simulink model "SR26"  (R2025a)
settings: Solver=FixedStepDiscrete  StartTime=0.0  StopTime=100  FixedStep=0.01  RelTol=1e-3  EnableMultiTasking=on
PreLoadFcn:
  | try, model_open; catch, disp('Error occurred while executing model pre-load callback: model_open.m'); disp('Please assure that the MATLAB working directory is set to the model directory before opening.'); end
InitFcn:
  | try, model_open; catch, end
values from neighbouring files (symbols this model uses):
  dt = 10.0    [SR26.sldd]
undefined symbols (not defined in the file or in its folder): BMSInputProcessing, GCM, raptor_get_safe_string, raptor_xcp_function, RegenEnable, StateCAN, Subsystem, TCEnable
libraries: Utilities x263, Raptor_lib x137, simulink x7, IO x5, APPS_BSPC x4, TorqueCommand x3, Cooling x3, StateMachine x2, DriveSpeed x2, ATCC x2, BrakePressure x2, ThrottlePosition x2
(part 3 of 4)

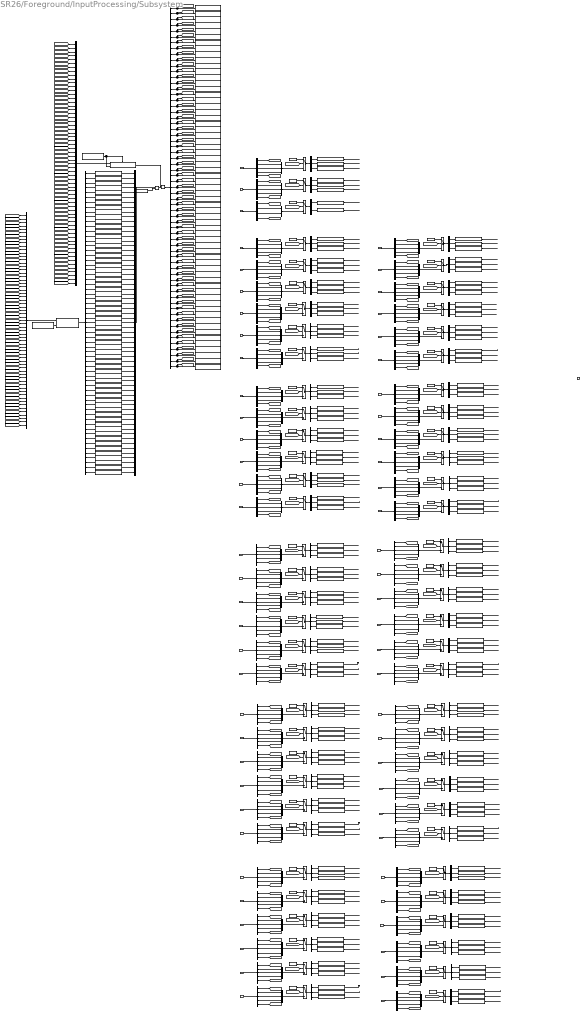
== system SR26/Foreground/InputProcessing/Subsystem ==
  note: Module5
  note: Module4
  note: Module3
  note: Module2
  note: 'IN_module2Cell4V_V'
  note: Module1
  note: times out after 200ms
  IO_CAN2_500_Bus : Inport
  IO_CAN2_501_Bus : Inport  Port=2
  IO_CAN2_502_Bus : Inport  Port=3
  IO_CAN2_503_Bus : Inport  Port=4
  IO_CAN2_504_Bus : Inport  Port=5
  IO_CAN2_505_Bus : Inport  Port=6
  IO_CAN2_506_Bus : Inport  Port=7
  IO_CAN2_507_Bus : Inport  Port=8
  IO_CAN2_508_Bus : Inport  Port=9
  IO_CAN2_509_Bus : Inport  Port=10
  IO_CAN2_510_Bus : Inport  Port=11
  IO_CAN2_511_Bus : Inport  Port=12
  IO_CAN2_512_Bus : Inport  Port=13
  IO_CAN2_513_Bus : Inport  Port=14
  IO_CAN2_514_Bus : Inport  Port=15
  IO_CAN2_515_Bus : Inport  Port=16
  IO_CAN2_516_Bus : Inport  Port=17
  IO_CAN2_517_Bus : Inport  Port=18
  IO_CAN2_518_Bus : Inport  Port=19
  IO_CAN2_519_Bus : Inport  Port=20
  IO_CAN2_520_Bus : Inport  Port=21
  IO_CAN2_521_Bus : Inport  Port=22
  IO_CAN2_522_Bus : Inport  Port=23
  IO_CAN2_523_Bus : Inport  Port=24
  IO_CAN2_524_Bus : Inport  Port=25
  IO_CAN2_525_Bus : Inport  Port=26
  IO_CAN2_526_Bus : Inport  Port=27
  IO_CAN2_527_Bus : Inport  Port=28
  IO_CAN2_528_Bus : Inport  Port=29
  IO_CAN2_529_Bus : Inport  Port=30
  IO_CAN2_530_Bus : Inport  Port=31
  IO_CAN2_531_Bus : Inport  Port=32
  IO_CAN2_532_Bus : Inport  Port=33
  IO_CAN2_533_Bus : Inport  Port=34
  IO_CAN2_534_Bus : Inport  Port=35
  IO_CAN2_535_Bus : Inport  Port=36
  IO_CAN2_536_Bus : Inport  Port=37
  IO_CAN2_537_Bus : Inport  Port=38
  IO_CAN2_538_Bus : Inport  Port=39
  IO_CAN2_539_Bus : Inport  Port=40
  IO_CAN2_540_Bus : Inport  Port=41
  IO_CAN2_541_Bus : Inport  Port=42
  IO_CAN2_542_Bus : Inport  Port=43
  IO_CAN2_543_Bus : Inport  Port=44
  IO_CAN2_544_Bus : Inport  Port=45
  IO_CAN2_545_Bus : Inport  Port=46
  IO_CAN2_546_Bus : Inport  Port=47
  IO_CAN2_547_Bus : Inport  Port=48
  IO_CAN2_548_Bus : Inport  Port=49
  IO_CAN2_549_Bus : Inport  Port=50
  IO_CAN2_550_Bus : Inport  Port=51
  IO_CAN2_551_Bus : Inport  Port=52
  IO_CAN2_552_Bus : Inport  Port=53
  IO_CAN2_553_Bus : Inport  Port=54
  IO_CAN2_554_Bus : Inport  Port=55
  IO_CAN2_555_Bus : Inport  Port=56
  IO_CAN2_556_Bus : Inport  Port=57
  IO_CAN2_557_Bus : Inport  Port=58
  IO_CAN2_558_Bus : Inport  Port=59
  IO_CAN2_559_Bus : Inport  Port=60
  IO_CAN2_560_Bus : Inport  Port=61
  IO_CAN2_561_Bus : Inport  Port=62
  In63 : Inport  Port=63
  Bus Selector : BusSelector  OutputSignals=Age,BMS_packCurr,BMS_packSOC,BMS_packVoltage,BMS_rollingMsg500
  Bus Selector1 : BusSelector  OutputSignals=Age,BMS_module1V,BMS_module2V,BMS_module3V,BMS_counterMsg501
  Bus Selector10 : BusSelector  OutputSignals=Age,BMS_module4Cell1Volt,BMS_module4Cell2Volt,BMS_module4Cell3Volt,BMS_counterMsg539
  Bus Selector11 : BusSelector  OutputSignals=Age,BMS_module1Cell7Temp,BMS_module1Cell8Temp,BMS_module1Cell9Temp,BMS_counterMsg511
  Bus Selector12 : BusSelector  OutputSignals=Age,BMS_module1Cell10Temp,BMS_module1Cell11Temp,BMS_module1Cell12Temp,BMS_counterMsg512
  Bus Selector13 : BusSelector  OutputSignals=Age,BMS_module1Cell16Temp,BMS_module1Cell17Temp,BMS_module1Cell18Temp,BMS_counterMsg514
  Bus Selector14 : BusSelector  OutputSignals=Age,BMS_module1Cell10Temp,BMS_module1Cell11Temp,BMS_module1Cell12Temp,BMS_counterMsg512
  Bus Selector15 : BusSelector  OutputSignals=Age,BMS_module2seg1V,BMS_module2seg2V,BMS_module2seg3V,BMS_counterMsg515
  Bus Selector16 : BusSelector  OutputSignals=Age,BMS_module2seg4V,BMS_module2seg5V,BMS_module2seg6V,BMS_counterMsg516
  Bus Selector17 : BusSelector  OutputSignals=Age,BMS_module1seg7V,BMS_module1seg8V,BMS_module1seg9V,BMS_counterMsg504
  Bus Selector18 : BusSelector  OutputSignals=Age,BMS_module2seg10V,BMS_module2seg11V,BMS_module2seg12V,BMS_counterMsg518
  Bus Selector19 : BusSelector  OutputSignals=Age,BMS_module2seg13V,BMS_module2seg14V,BMS_module2seg15V,BMS_counterMsg519
  Bus Selector2 : BusSelector  OutputSignals=Age,BMS_module4V,BMS_module5V,BMS_counterMsg502
  Bus Selector20 : BusSelector  OutputSignals=Age,BMS_module2seg16V,BMS_module2seg17V,BMS_module2seg18V,BMS_counterMsg520
  Bus Selector21 : BusSelector  OutputSignals=Age,BMS_module2Cell4Temp,BMS_module2Cell5Temp,BMS_module2Cell6Temp,BMS_counterMsg522
  Bus Selector22 : BusSelector  OutputSignals=Age,BMS_module2Cell7Temp,BMS_module2Cell8Temp,BMS_module2Cell9Temp,BMS_counterMsg523
  Bus Selector23 : BusSelector  OutputSignals=Age,BMS_module2Cell10Temp,BMS_module2Cell11Temp,BMS_module2Cell12Temp,BMS_counterMsg524
  Bus Selector24 : BusSelector  OutputSignals=Age,BMS_module2Cell16Temp,BMS_module2Cell17Temp,BMS_module2Cell18Temp,BMS_counterMsg526
  Bus Selector25 : BusSelector  OutputSignals=Age,BMS_module2Cell13Temp,BMS_module2Cell14Temp,BMS_module2Cell15Temp,BMS_counterMsg525
  Bus Selector26 : BusSelector  OutputSignals=Age,BMS_module3seg1V,BMS_module3seg2V,BMS_module3seg3V,BMS_counterMsg527
  Bus Selector27 : BusSelector  OutputSignals=Age,BMS_module2Cell1Temp,BMS_module2Cell2Temp,BMS_module2Cell3Temp,BMS_counterMsg521
  Bus Selector28 : BusSelector  OutputSignals=Age,BMS_module3Cell4Volt,BMS_module3Cell5Volt,BMS_module3Cell6Volt,BMS_counterMsg528
  Bus Selector29 : BusSelector  OutputSignals=Age,BMS_module3Cell7Volt,BMS_module3Cell8Volt,BMS_module3Cell9Volt,BMS_counterMsg529
  Bus Selector3 : BusSelector  OutputSignals=Age,BMS_module1Cell1Volt,BMS_module1Cell2Volt,BMS_module1Cell3Volt,BMS_counterMsg503
  Bus Selector30 : BusSelector  OutputSignals=Age,BMS_module3Cell10Volt,BMS_module3Cell11Volt,BMS_module3Cell12Volt,BMS_counterMsg530
  Bus Selector31 : BusSelector  OutputSignals=Age,BMS_module3seg13V,BMS_module3seg14V,BMS_module3seg15V,BMS_counterMsg531
  Bus Selector32 : BusSelector  OutputSignals=Age,BMS_module3seg16V,BMS_module3seg17V,BMS_module3seg18V,BMS_counterMsg532
  Bus Selector33 : BusSelector  OutputSignals=Age,BMS_module3Cell4Temp,BMS_module3Cell5Temp,BMS_module3Cell6Temp,BMS_counterMsg534
  Bus Selector34 : BusSelector  OutputSignals=Age,BMS_module3Cell7Temp,BMS_module3Cell8Temp,BMS_module3Cell9Temp,BMS_counterMsg535
  Bus Selector35 : BusSelector  OutputSignals=Age,BMS_module3Cell10Temp,BMS_module3Cell11Temp,BMS_module3Cell12Temp,BMS_counterMsg536
  Bus Selector36 : BusSelector  OutputSignals=Age,BMS_module3Cell16Temp,BMS_module3Cell17Temp,BMS_module3Cell18Temp,BMS_counterMsg538
  Bus Selector37 : BusSelector  OutputSignals=Age,BMS_module3Cell13Temp,BMS_module3Cell14Temp,BMS_module3Cell15Temp,BMS_counterMsg537
  Bus Selector38 : BusSelector  OutputSignals=Age,BMS_module3Cell1Temp,BMS_module3Cell2Temp,BMS_module3Cell3Temp,BMS_counterMsg533
  Bus Selector39 : BusSelector  OutputSignals=Age,BMS_module1Cell4Temp,BMS_module1Cell5Temp,BMS_module1Cell6Temp,BMS_counterMsg510
  Bus Selector4 : BusSelector  OutputSignals=Age,BMS_module1Cell4Volt,BMS_module1Cell5Volt,BMS_module1Cell6Volt,BMS_counterMsg504
  Bus Selector40 : BusSelector  OutputSignals=Age,BMS_module4Cell4Volt,BMS_module4Cell5Volt,BMS_module4Cell6Volt,BMS_counterMsg540
  Bus Selector41 : BusSelector  OutputSignals=Age,BMS_module4Cell7Volt,BMS_module4Cell8Volt,BMS_module4Cell9Volt,BMS_counterMsg541
  Bus Selector42 : BusSelector  OutputSignals=Age,BMS_module4Cell10Volt,BMS_module4Cell11Volt,BMS_module4Cell12Volt,BMS_counterMsg542
  Bus Selector43 : BusSelector  OutputSignals=Age,BMS_module4Cell13Volt,BMS_module4Cell14Volt,BMS_module4Cell15Volt,BMS_counterMsg543
  Bus Selector44 : BusSelector  OutputSignals=Age,BMS_module4Cell16Volt,BMS_module4Cell17Volt,BMS_module4Cell18Volt,BMS_counterMsg544
  Bus Selector45 : BusSelector  OutputSignals=Age,BMS_module4Cell4Temp,BMS_module4Cell5Temp,BMS_module4Cell6Temp,BMS_counterMsg546
  Bus Selector46 : BusSelector  OutputSignals=Age,BMS_module4Cell7Temp,BMS_module4Cell8Temp,BMS_module4Cell9Temp,BMS_counterMsg547
  Bus Selector47 : BusSelector  OutputSignals=Age,BMS_module4Cell10Temp,BMS_module4Cell11Temp,BMS_module4Cell12Temp,BMS_counterMsg548
  Bus Selector48 : BusSelector  OutputSignals=Age,BMS_module4Cell16Temp,BMS_module4Cell17Temp,BMS_module4Cell18Temp,BMS_counterMsg550
  Bus Selector49 : BusSelector  OutputSignals=Age,BMS_module4Cell13Temp,BMS_module4Cell14Temp,BMS_module4Cell15Temp,BMS_counterMsg549
  Bus Selector5 : BusSelector  OutputSignals=Age,BMS_module1Cell7Volt,BMS_module1Cell8Volt,BMS_module1Cell9Volt,BMS_counterMsg505
  Bus Selector50 : BusSelector  OutputSignals=Age,BMS_module4Cell1Temp,BMS_module4Cell2Temp,BMS_module4Cell3Temp,BMS_counterMsg545
  Bus Selector51 : BusSelector  OutputSignals=Age,BMS_module5Cell1Volt,BMS_module5Cell2Volt,BMS_module5Cell3Volt,BMS_counterMsg551
  Bus Selector52 : BusSelector  OutputSignals=Age,BMS_module5Cell4Volt,BMS_module5Cell5Volt,BMS_module5Cell6Volt,BMS_counterMsg552
  Bus Selector53 : BusSelector  OutputSignals=Age,BMS_module5Cell7Volt,BMS_module5Cell8Volt,BMS_module5Cell9Volt,BMS_counterMsg553
  Bus Selector54 : BusSelector  OutputSignals=Age,BMS_module5Cell10Volt,BMS_module5Cell11Volt,BMS_module5Cell12Volt,BMS_counterMsg554
  Bus Selector55 : BusSelector  OutputSignals=Age,BMS_module5Cell13Volt,BMS_module5Cell14Volt,BMS_module5Cell15Volt,BMS_counterMsg555
  Bus Selector56 : BusSelector  OutputSignals=Age,BMS_module5Cell16Volt,BMS_module5Cell17Volt,BMS_module5Cell18Volt,BMS_counterMsg556
  Bus Selector57 : BusSelector  OutputSignals=Age,BMS_module5Cell4Temp,BMS_module5Cell5Temp,BMS_module5Cell6Temp,BMS_counterMsg558
  Bus Selector58 : BusSelector  OutputSignals=Age,BMS_module5Cell7Temp,BMS_module5Cell8Temp,BMS_module5Cell9Temp,BMS_counterMsg559
  Bus Selector59 : BusSelector  OutputSignals=Age,BMS_module5Cell10Temp,BMS_module5Cell11Temp,BMS_module5Cell12Temp,BMS_counterMsg560
  Bus Selector6 : BusSelector  OutputSignals=Age,BMS_module1Cell10Volt,BMS_module1Cell11Volt,BMS_module1Cell12Volt,BMS_counterMsg506
  Bus Selector60 : BusSelector  OutputSignals=Age,BMS_module5Cell16Temp,BMS_module5Cell17Temp,BMS_module5Cell18Temp,BMS_counterMsg562
  Bus Selector61 : BusSelector  OutputSignals=Age,BMS_module5Cell13Temp,BMS_module5Cell14Temp,BMS_module5Cell15Temp,BMS_counterMsg561
  Bus Selector62 : BusSelector  OutputSignals=Age,BMS_module5Cell1Temp,BMS_module5Cell2Temp,BMS_module5Cell3Temp,BMS_counterMsg557
  Bus Selector7 : BusSelector  OutputSignals=Age,BMS_module1Cell13Volt,BMS_module1Cell14Volt,BMS_module1Cell15Volt,BMS_counterMsg507
  Bus Selector8 : BusSelector  OutputSignals=Age,BMS_module1Cell16Volt,BMS_module1Cell17Volt,BMS_module1Cell18Volt,BMS_counterMsg508
  Bus Selector9 : BusSelector  OutputSignals=Age,BMS_module1Cell1Temp,BMS_module1Cell2Temp,BMS_module1Cell3Temp,BMS_counterMsg509
  CANTimeoutCheck : Utilities/CANTimeoutCheck
  Constant{,1..62} (63 alike) : Constant  Value=int16(32767)
  Demux : Demux  Outputs=63
  Demux1 : Demux  Outputs=63
  Demux{2..3,5..64} (62 alike) : Demux  Outputs=3
  Demux4 : Demux  Outputs=2
  Enumerated Constant : simulink/Sources/Enumerated Constant  OutDataTypeStr=Enum: StateCAN  Value=StateCAN.Normal  SampleTime=inf
  EnumeratedOverMeas{,3,8,11,16,19,25,30,32,35,40,43,50,55..56,62} (16 alike) : Utilities/EnumeratedOverMeas  sigName='IN_CAN1_301_Status_en'  enumName='StateCAN'
  EnumeratedOverMeas{1,5,9,13,17,21,27,31,33,37,41,46,52,57,59,63} (16 alike) : Utilities/EnumeratedOverMeas  sigName='IN_CAN1_302_Status_en'  enumName='StateCAN'
  EnumeratedOverMeas{2,6,10,14,18,22,24,28,34,38,42,44,47,49,53,60} (16 alike) : Utilities/EnumeratedOverMeas  sigName='IN_CAN1_303_Staus_en'  enumName='StateCAN'
  EnumeratedOverMeas{4,7,12,15,20,23,26,29,36,39,45,51,54,58,61} (15 alike) : Utilities/EnumeratedOverMeas  sigName='IN_CAN1_305_Status_en'  enumName='StateCAN'
  Equal : RelationalOperator  Operator=~=  OutDataTypeStr=boolean  RndMeth=Simplest  InputSameDT=off
  Logical Operator : Logic  Operator=OR  AllPortsSameDT=off  OutDataTypeStr=boolean
  Mux : Mux  Inputs=63
  Mux1 : Mux  Inputs=63
  Mux{3..4,6..65} (62 alike) : Mux  Inputs=3
  Mux2 : Mux  Inputs=63
  Mux5 : Mux  Inputs=2
  OverMeas : Utilities/OverMeas  sigName='IN_PackCurrent_A'  minimum=-inf  maximum=inf
  OverMeas1 : Utilities/OverMeas  sigName='IN_PackSOC_pct'  minimum=-inf  maximum=inf
  OverMeas10 : Utilities/OverMeas  sigName='IN_module1Cell2Volt_V'  minimum=-inf  maximum=inf
  OverMeas100 : Utilities/OverMeas  sigName='IN_module3Cell2Temp_degC'  minimum=-inf  maximum=inf
  OverMeas101 : Utilities/OverMeas  sigName='IN_module3Cell3Temp_degC'  minimum=-inf  maximum=inf
  OverMeas102 : Utilities/OverMeas  sigName='IN_module3Cell4Temp_degC'  minimum=-inf  maximum=inf
  OverMeas103 : Utilities/OverMeas  sigName='IN_module3Cell5Temp_degC'  minimum=-inf  maximum=inf
  OverMeas104 : Utilities/OverMeas  sigName='IN_module3Cell6Temp_degC'  minimum=-inf  maximum=inf
  OverMeas105 : Utilities/OverMeas  sigName='IN_module3Cell7Temp_degC'  minimum=-inf  maximum=inf
  OverMeas106 : Utilities/OverMeas  sigName='IN_module3Cell8Temp_degC'  minimum=-inf  maximum=inf
  OverMeas107 : Utilities/OverMeas  sigName='IN_module3Cell9Temp_degC'  minimum=-inf  maximum=inf
  OverMeas108 : Utilities/OverMeas  sigName='IN_module3Cell13Temp_degC'  minimum=-inf  maximum=inf
  OverMeas109 : Utilities/OverMeas  sigName='IN_module3Cell10Temp_degC'  minimum=-inf  maximum=inf
  OverMeas11 : Utilities/OverMeas  sigName='IN_module1Cell3Volt_V'  minimum=-inf  maximum=inf
  OverMeas110 : Utilities/OverMeas  sigName='IN_module3Cell11Temp_degC'  minimum=-inf  maximum=inf
  OverMeas111 : Utilities/OverMeas  sigName='IN_module3Cell14Temp_degC'  minimum=-inf  maximum=inf
  OverMeas112 : Utilities/OverMeas  sigName='IN_module3Cell12Temp_degC'  minimum=-inf  maximum=inf
  OverMeas113 : Utilities/OverMeas  sigName='IN_module3Cell15Temp_degC'  minimum=-inf  maximum=inf
  OverMeas114 : Utilities/OverMeas  sigName='IN_module3Cell17Temp_degC'  minimum=-inf  maximum=inf
  OverMeas115 : Utilities/OverMeas  sigName='IN_module3Cell18Temp_degC'  minimum=-inf  maximum=inf
  OverMeas116 : Utilities/OverMeas  sigName='IN_module4Cell2V_V'  minimum=-inf  maximum=inf
  OverMeas117 : Utilities/OverMeas  sigName='IN_module4Cell3V_V'  minimum=-inf  maximum=inf
  OverMeas118 : Utilities/OverMeas  sigName='IN_module4Cell1V_V'  minimum=-inf  maximum=inf
  OverMeas119 : Utilities/OverMeas  sigName='IN_module4Cell4V_V'  minimum=-inf  maximum=inf
  OverMeas12 : Utilities/OverMeas  sigName='IN_module1Cell4Volt_V'  minimum=-inf  maximum=inf
  OverMeas120 : Utilities/OverMeas  sigName='IN_module4Cell5V_V'  minimum=-inf  maximum=inf
  OverMeas121 : Utilities/OverMeas  sigName='IN_module4Cell6V_V'  minimum=-inf  maximum=inf
  OverMeas122 : Utilities/OverMeas  sigName='IN_module4Cell7V_V'  minimum=-inf  maximum=inf
  OverMeas123 : Utilities/OverMeas  sigName='IN_module4Cell8V_V'  minimum=-inf  maximum=inf
  OverMeas124 : Utilities/OverMeas  sigName='IN_module4Cell9V_V'  minimum=-inf  maximum=inf
  OverMeas125 : Utilities/OverMeas  sigName='IN_module4Cell15V_V'  minimum=-inf  maximum=inf
  OverMeas126 : Utilities/OverMeas  sigName='IN_module4Cell17V_V'  minimum=-inf  maximum=inf
  OverMeas127 : Utilities/OverMeas  sigName='IN_module4Cell18V_V'  minimum=-inf  maximum=inf
  OverMeas128 : Utilities/OverMeas  sigName='IN_module4Cell10V_V'  minimum=-inf  maximum=inf
  OverMeas129 : Utilities/OverMeas  sigName='IN_module4Cell11V_V'  minimum=-inf  maximum=inf
  OverMeas13 : Utilities/OverMeas  sigName='IN_module1Cell5Volt_V'  minimum=-inf  maximum=inf
  OverMeas130 : Utilities/OverMeas  sigName='IN_module4Cell13V_V'  minimum=-inf  maximum=inf
  OverMeas131 : Utilities/OverMeas  sigName='IN_module4Cell12V_V'  minimum=-inf  maximum=inf
  OverMeas132 : Utilities/OverMeas  sigName='IN_module4Cell14V_V'  minimum=-inf  maximum=inf
  OverMeas133 : Utilities/OverMeas  sigName='IN_module4Cell16V_V'  minimum=-inf  maximum=inf
  OverMeas134 : Utilities/OverMeas  sigName='IN_module4Cell2Temp_degC'  minimum=-inf  maximum=inf
  OverMeas135 : Utilities/OverMeas  sigName='IN_module4Cell3Temp_degC'  minimum=-inf  maximum=inf
  OverMeas136 : Utilities/OverMeas  sigName='IN_module4Cell4Temp_degC'  minimum=-inf  maximum=inf
  OverMeas137 : Utilities/OverMeas  sigName='IN_module4Cell5Temp_degC'  minimum=-inf  maximum=inf
  OverMeas138 : Utilities/OverMeas  sigName='IN_module4Cell6Temp_degC'  minimum=-inf  maximum=inf
  OverMeas139 : Utilities/OverMeas  sigName='IN_module4Cell7Temp_degC'  minimum=-inf  maximum=inf
  OverMeas14 : Utilities/OverMeas  sigName='IN_module1Cell6Volt_V'  minimum=-inf  maximum=inf
  OverMeas140 : Utilities/OverMeas  sigName='IN_module4Cell8Temp_degC'  minimum=-inf  maximum=inf
  OverMeas141 : Utilities/OverMeas  sigName='IN_module4Cell9Temp_degC'  minimum=-inf  maximum=inf
  OverMeas142 : Utilities/OverMeas  sigName='IN_modul4Cell13Temp_degC'  minimum=-inf  maximum=inf
  OverMeas143 : Utilities/OverMeas  sigName='IN_module4Cell10Temp_degC'  minimum=-inf  maximum=inf
  OverMeas144 : Utilities/OverMeas  sigName='IN_module4Cell11Temp_degC'  minimum=-inf  maximum=inf
  OverMeas145 : Utilities/OverMeas  sigName='IN_module4Cell14Temp_degC'  minimum=-inf  maximum=inf
  OverMeas146 : Utilities/OverMeas  sigName='IN_module4Cell12Temp_degC'  minimum=-inf  maximum=inf
  OverMeas147 : Utilities/OverMeas  sigName='IN_module4Cell15Temp_degC'  minimum=-inf  maximum=inf
  OverMeas148 : Utilities/OverMeas  sigName='IN_module4Cell17Temp_degC'  minimum=-inf  maximum=inf
  OverMeas149 : Utilities/OverMeas  sigName='IN_module4Cell18Temp_degC'  minimum=-inf  maximum=inf
  OverMeas15 : Utilities/OverMeas  sigName='IN_module1Cell7Volt_V'  minimum=-inf  maximum=inf
  OverMeas150 : Utilities/OverMeas  sigName='IN_module4Cell16Temp_degC'  minimum=-inf  maximum=inf
  OverMeas151 : Utilities/OverMeas  sigName='IN_module4Cell1Temp_degC'  minimum=-inf  maximum=inf
  OverMeas152 : Utilities/OverMeas  sigName='IN_module5Cell2V_V'  minimum=-inf  maximum=inf
  OverMeas153 : Utilities/OverMeas  sigName='IN_module5Cell3V_V'  minimum=-inf  maximum=inf
  OverMeas154 : Utilities/OverMeas  sigName='IN_module5Cell1V_V'  minimum=-inf  maximum=inf
  OverMeas155 : Utilities/OverMeas  sigName='IN_module5Cell4V_V'  minimum=-inf  maximum=inf
  OverMeas156 : Utilities/OverMeas  sigName='IN_module5Cell5V_V'  minimum=-inf  maximum=inf
  OverMeas157 : Utilities/OverMeas  sigName='IN_module5Cell6V_V'  minimum=-inf  maximum=inf
  OverMeas158 : Utilities/OverMeas  sigName='IN_module5Cell7V_V'  minimum=-inf  maximum=inf
  OverMeas159 : Utilities/OverMeas  sigName='IN_module5Cell8V_V'  minimum=-inf  maximum=inf
  OverMeas16 : Utilities/OverMeas  sigName='IN_module1Cell8Volt_V'  minimum=-inf  maximum=inf
  OverMeas160 : Utilities/OverMeas  sigName='IN_module4Cell9V_V'  minimum=-inf  maximum=inf
  OverMeas161 : Utilities/OverMeas  sigName='IN_module5Cell15V_V'  minimum=-inf  maximum=inf
  OverMeas162 : Utilities/OverMeas  sigName='IN_module5Cell17V_V'  minimum=-inf  maximum=inf
  OverMeas163 : Utilities/OverMeas  sigName='IN_module5Cell18V_V'  minimum=-inf  maximum=inf
  OverMeas164 : Utilities/OverMeas  sigName='IN_module5Cell10V_V'  minimum=-inf  maximum=inf
  OverMeas165 : Utilities/OverMeas  sigName='IN_module5Cell11V_V'  minimum=-inf  maximum=inf
  OverMeas166 : Utilities/OverMeas  sigName='IN_module5Cell13V_V'  minimum=-inf  maximum=inf
  OverMeas167 : Utilities/OverMeas  sigName='IN_module5Cell12V_V'  minimum=-inf  maximum=inf
  OverMeas168 : Utilities/OverMeas  sigName='IN_module5Cell14V_V'  minimum=-inf  maximum=inf
  OverMeas169 : Utilities/OverMeas  sigName='IN_module5Cell16V_V'  minimum=-inf  maximum=inf
  OverMeas17 : Utilities/OverMeas  sigName='IN_module1Cell9Volt_V'  minimum=-inf  maximum=inf
  OverMeas170 : Utilities/OverMeas  sigName='IN_module4Cell2Temp_degC'  minimum=-inf  maximum=inf
  OverMeas171 : Utilities/OverMeas  sigName='IN_module4Cell3Temp_degC'  minimum=-inf  maximum=inf
  OverMeas172 : Utilities/OverMeas  sigName='IN_module4Cell4Temp_degC'  minimum=-inf  maximum=inf
  OverMeas173 : Utilities/OverMeas  sigName='IN_module4Cell5Temp_degC'  minimum=-inf  maximum=inf
  OverMeas174 : Utilities/OverMeas  sigName='IN_module4Cell6Temp_degC'  minimum=-inf  maximum=inf
  OverMeas175 : Utilities/OverMeas  sigName='IN_module5Cell7Temp_degC'  minimum=-inf  maximum=inf
  OverMeas176 : Utilities/OverMeas  sigName='IN_module5Cell8Temp_degC'  minimum=-inf  maximum=inf
  OverMeas177 : Utilities/OverMeas  sigName='IN_module5Cell9Temp_degC'  minimum=-inf  maximum=inf
  OverMeas178 : Utilities/OverMeas  sigName='IN_module5Cell13Temp_degC'  minimum=-inf  maximum=inf
  OverMeas179 : Utilities/OverMeas  sigName='IN_module5Cell10Temp_degC'  minimum=-inf  maximum=inf
  OverMeas18 : Utilities/OverMeas  sigName='IN_module1Cell15Volt_V'  minimum=-inf  maximum=inf
  OverMeas180 : Utilities/OverMeas  sigName='IN_module5Cell11Temp_degC'  minimum=-inf  maximum=inf
  OverMeas181 : Utilities/OverMeas  sigName='IN_module5Cell14Temp_degC'  minimum=-inf  maximum=inf
  OverMeas182 : Utilities/OverMeas  sigName='IN_module5Cell12Temp_degC'  minimum=-inf  maximum=inf
  OverMeas183 : Utilities/OverMeas  sigName='IN_module5Cell15Temp_degC'  minimum=-inf  maximum=inf
  OverMeas184 : Utilities/OverMeas  sigName='IN_module5Cell17Temp_degC'  minimum=-inf  maximum=inf
  OverMeas185 : Utilities/OverMeas  sigName='IN_module5Cell18Temp_degC'  minimum=-inf  maximum=inf
  OverMeas186 : Utilities/OverMeas  sigName='IN_module5Cell16Temp_degC'  minimum=-inf  maximum=inf
  OverMeas187 : Utilities/OverMeas  sigName='IN_module4Cell1Temp_degC'  minimum=-inf  maximum=inf
  OverMeas19 : Utilities/OverMeas  sigName='IN_module1Cell17V_V'  minimum=-inf  maximum=inf
  OverMeas2 : Utilities/OverMeas  sigName='IN_PackVoltage_V'  minimum=-inf  maximum=inf
  OverMeas20 : Utilities/OverMeas  sigName='IN_module1Cell18V_V'  minimum=-inf  maximum=inf
  OverMeas21 : Utilities/OverMeas  sigName='IN_module1Cell16Temp_degC'  minimum=-inf  maximum=inf
  OverMeas22 : Utilities/OverMeas  sigName='IN_module1Cell1Temp_degC'  minimum=-inf  maximum=inf
  OverMeas23 : Utilities/OverMeas  sigName='IN_module1Cell2Temp_degC'  minimum=-inf  maximum=inf
  OverMeas24 : Utilities/OverMeas  sigName='IN_module1Cell3Temp_degC'  minimum=-inf  maximum=inf
  OverMeas25 : Utilities/OverMeas  sigName='IN_module1Cell10Volt_V'  minimum=-inf  maximum=inf
  OverMeas26 : Utilities/OverMeas  sigName='IN_module1Cell11Volt_V'  minimum=-inf  maximum=inf
  OverMeas27 : Utilities/OverMeas  sigName='IN_module1Cell13Volt_V'  minimum=-inf  maximum=inf
  OverMeas28 : Utilities/OverMeas  sigName='IN_module1Cell12Volt_V'  minimum=-inf  maximum=inf
  OverMeas29 : Utilities/OverMeas  sigName='IN_module1Cell4Temp_degC'  minimum=-inf  maximum=inf
  OverMeas3 : Utilities/OverMeas  sigName='IN_module1V_V'  minimum=-inf  maximum=inf
  OverMeas30 : Utilities/OverMeas  sigName='IN_module1Cell5Temp_degC'  minimum=-inf  maximum=inf
  OverMeas31 : Utilities/OverMeas  sigName='IN_module1Cell6Temp_degC'  minimum=-inf  maximum=inf
  OverMeas32 : Utilities/OverMeas  sigName='IN_module1Cell7Temp_degC'  minimum=-inf  maximum=inf
  OverMeas33 : Utilities/OverMeas  sigName='IN_module1Cell8Temp_degC'  minimum=-inf  maximum=inf
  OverMeas34 : Utilities/OverMeas  sigName='IN_module1Cell9Temp_degC'  minimum=-inf  maximum=inf
  OverMeas35 : Utilities/OverMeas  sigName='IN_module1Cell13Temp_degC'  minimum=-inf  maximum=inf
  OverMeas36 : Utilities/OverMeas  sigName='IN_module1Cell10Temp_degC'  minimum=-inf  maximum=inf
  OverMeas37 : Utilities/OverMeas  sigName='IN_module1Cell11Temp_degC'  minimum=-inf  maximum=inf
  OverMeas38 : Utilities/OverMeas  sigName='IN_module1Cell14Temp_degC'  minimum=-inf  maximum=inf
  OverMeas39 : Utilities/OverMeas  sigName='IN_module1Cell12Temp_degC'  minimum=-inf  maximum=inf
  OverMeas4 : Utilities/OverMeas  sigName='IN_module2V_V'  minimum=-inf  maximum=inf
  OverMeas40 : Utilities/OverMeas  sigName='IN_module1Cell15Temp_degC'  minimum=-inf  maximum=inf
  OverMeas41 : Utilities/OverMeas  sigName='IN_module1Cell17Temp_degC'  minimum=-inf  maximum=inf
  OverMeas42 : Utilities/OverMeas  sigName='IN_module2Cell2V_V'  minimum=-inf  maximum=inf
  OverMeas43 : Utilities/OverMeas  sigName='IN_module2Cell3V_V'  minimum=-inf  maximum=inf
  OverMeas44 : Utilities/OverMeas  sigName='IN_module2Cell4V_V'  minimum=-inf  maximum=inf
  OverMeas45 : Utilities/OverMeas  sigName='IN_module2Cell5V_V'  minimum=-inf  maximum=inf
  OverMeas46 : Utilities/OverMeas  sigName='IN_module2Cell6V_V'  minimum=-inf  maximum=inf
  OverMeas47 : Utilities/OverMeas  sigName='IN_module2Cell7V_V'  minimum=-inf  maximum=inf
  OverMeas48 : Utilities/OverMeas  sigName='IN_module2Cell8V_V'  minimum=-inf  maximum=inf
  OverMeas49 : Utilities/OverMeas  sigName='IN_module2Cell9V_V'  minimum=-inf  maximum=inf
  OverMeas5 : Utilities/OverMeas  sigName='IN_module3V_V'  minimum=-inf  maximum=inf
  OverMeas50 : Utilities/OverMeas  sigName='IN_module2Cell15V_V'  minimum=-inf  maximum=inf
  OverMeas51 : Utilities/OverMeas  sigName='IN_module2Cell17V_V'  minimum=-inf  maximum=inf
  OverMeas52 : Utilities/OverMeas  sigName='IN_module2Cell18V_V'  minimum=-inf  maximum=inf
  OverMeas53 : Utilities/OverMeas  sigName='IN_module2Cell10V_V'  minimum=-inf  maximum=inf
  OverMeas54 : Utilities/OverMeas  sigName='IN_module2Cell11V_V'  minimum=-inf  maximum=inf
  OverMeas55 : Utilities/OverMeas  sigName='IN_module2Cell13V_V'  minimum=-inf  maximum=inf
  OverMeas56 : Utilities/OverMeas  sigName='IN_module2Cell12V_V'  minimum=-inf  maximum=inf
  OverMeas57 : Utilities/OverMeas  sigName='IN_module2Cell14V_V'  minimum=-inf  maximum=inf
  OverMeas58 : Utilities/OverMeas  sigName='IN_module2Cell1V_V'  minimum=-inf  maximum=inf
  OverMeas59 : Utilities/OverMeas  sigName='IN_module1Cell18Temp_degC'  minimum=-inf  maximum=inf
  OverMeas6 : Utilities/OverMeas  sigName='IN_module4V_V'  minimum=-inf  maximum=inf
  OverMeas60 : Utilities/OverMeas  sigName='IN_module2Cell16Temp_degC'  minimum=-inf  maximum=inf
  OverMeas61 : Utilities/OverMeas  sigName='IN_module2Cell1Temp_degC'  minimum=-inf  maximum=inf
  OverMeas62 : Utilities/OverMeas  sigName='IN_module2Cell2Temp_degC'  minimum=-inf  maximum=inf
  OverMeas63 : Utilities/OverMeas  sigName='IN_module2Cell3Temp_degC'  minimum=-inf  maximum=inf
  OverMeas64 : Utilities/OverMeas  sigName='IN_module2Cell4Temp_degC'  minimum=-inf  maximum=inf
  OverMeas65 : Utilities/OverMeas  sigName='IN_module2Cell5Temp_degC'  minimum=-inf  maximum=inf
  OverMeas66 : Utilities/OverMeas  sigName='IN_module2Cell6Temp_degC'  minimum=-inf  maximum=inf
  OverMeas67 : Utilities/OverMeas  sigName='IN_module2Cell7Temp_degC'  minimum=-inf  maximum=inf
  OverMeas68 : Utilities/OverMeas  sigName='IN_module2Cell8Temp_degC'  minimum=-inf  maximum=inf
  OverMeas69 : Utilities/OverMeas  sigName='IN_module2Cell9Temp_degC'  minimum=-inf  maximum=inf
  OverMeas7 : Utilities/OverMeas  sigName='IN_module5V_V'  minimum=-inf  maximum=inf
  OverMeas70 : Utilities/OverMeas  sigName='IN_module2Cell13Temp_degC'  minimum=-inf  maximum=inf
  OverMeas71 : Utilities/OverMeas  sigName='IN_module2Cell10Temp_degC'  minimum=-inf  maximum=inf
  OverMeas72 : Utilities/OverMeas  sigName='IN_module2Cell11Temp_degC'  minimum=-inf  maximum=inf
  OverMeas73 : Utilities/OverMeas  sigName='IN_module2Cell14Temp_degC'  minimum=-inf  maximum=inf
  OverMeas74 : Utilities/OverMeas  sigName='IN_module2Cell12Temp_degC'  minimum=-inf  maximum=inf
  OverMeas75 : Utilities/OverMeas  sigName='IN_module2Cell15Temp_degC'  minimum=-inf  maximum=inf
  OverMeas76 : Utilities/OverMeas  sigName='IN_module2Cell17Temp_degC'  minimum=-inf  maximum=inf
  OverMeas77 : Utilities/OverMeas  sigName='IN_module3Cell2V_V'  minimum=-inf  maximum=inf
  OverMeas78 : Utilities/OverMeas  sigName='IN_module3Cell3V_V'  minimum=-inf  maximum=inf
  OverMeas79 : Utilities/OverMeas  sigName='IN_module3Cell1V_V'  minimum=-inf  maximum=inf
  OverMeas8 : Utilities/OverMeas  sigName='IN_module1Cell14Volt_V'  minimum=-inf  maximum=inf
  OverMeas80 : Utilities/OverMeas  sigName='IN_module2Cell18Temp_degC'  minimum=-inf  maximum=inf
  OverMeas81 : Utilities/OverMeas  sigName='IN_module2Cell16V_V'  minimum=-inf  maximum=inf
  OverMeas82 : Utilities/OverMeas  sigName='IN_module3Cell4V_V'  minimum=-inf  maximum=inf
  OverMeas83 : Utilities/OverMeas  sigName='IN_module3Seg5V_V'  minimum=-inf  maximum=inf
  OverMeas84 : Utilities/OverMeas  sigName='IN_module3Seg6V_V'  minimum=-inf  maximum=inf
  OverMeas85 : Utilities/OverMeas  sigName='IN_module3Cell7V_V'  minimum=-inf  maximum=inf
  OverMeas86 : Utilities/OverMeas  sigName='IN_module3Cell8V_V'  minimum=-inf  maximum=inf
  OverMeas87 : Utilities/OverMeas  sigName='IN_module3Cell9V_V'  minimum=-inf  maximum=inf
  OverMeas88 : Utilities/OverMeas  sigName='IN_module3Cell15V_V'  minimum=-inf  maximum=inf
  OverMeas89 : Utilities/OverMeas  sigName='IN_module3Cell17V_V'  minimum=-inf  maximum=inf
  OverMeas9 : Utilities/OverMeas  sigName='IN_module1Cell1Volt_V'  minimum=-inf  maximum=inf
  OverMeas90 : Utilities/OverMeas  sigName='IN_module3Cell18V_V'  minimum=-inf  maximum=inf
  OverMeas91 : Utilities/OverMeas  sigName='IN_module3Cell10V_V'  minimum=-inf  maximum=inf
  OverMeas92 : Utilities/OverMeas  sigName='IN_module3Cell11V_V'  minimum=-inf  maximum=inf
  OverMeas93 : Utilities/OverMeas  sigName='IN_module3Cell13V_V'  minimum=-inf  maximum=inf
  OverMeas94 : Utilities/OverMeas  sigName='IN_module3Cell12V_V'  minimum=-inf  maximum=inf
  OverMeas95 : Utilities/OverMeas  sigName='IN_module3Cell14V_V'  minimum=-inf  maximum=inf
  OverMeas96 : Utilities/OverMeas  sigName='IN_module3Cell16V_V'  minimum=-inf  maximum=inf
  OverMeas97 : Utilities/OverMeas  sigName='IN_module1Cell16V_V'  minimum=-inf  maximum=inf
  OverMeas98 : Utilities/OverMeas  sigName='IN_module3Cell16Temp_degC'  minimum=-inf  maximum=inf
  OverMeas99 : Utilities/OverMeas  sigName='IN_module3Cell1Temp_degC'  minimum=-inf  maximum=inf
  RollingCounterCheck : Utilities/RollingCounterCheck
  Switch{,1..62} (63 alike) : Switch  Criteria=u2 > Threshold  SaturateOnIntegerOverflow=off  InputSameDT=off
  raptor_adjustment : Raptor_lib/Data Storage/raptor_adjustment  paramName='IN_BMSTOThresh_na'  nameSource=Parameter  initValue=20  dataType=int32  storage=Calibration  calDispType=Number  calEnum={'False', 'True'}  calGain=1.0  calOffset=0.0  calMax=inf  calMin=-inf  calFormat='-1'  calUnit=''  calHelp=''  calAccess=1  calFunction=raptor_xcp_function(gcb)  calDispHeaders=off  calColHeaders={'Col1' 'Col2' 'Col3'}  calRowHeaders={'Row1' 'Row2' 'Row3'}
      settings: SourceProductName=Raptor
  raptor_adjustment1 : Raptor_lib/Data Storage/raptor_adjustment  paramName='IN_BMSRollingCounterEnable'  nameSource=Parameter  initValue=1  dataType=boolean  storage=Calibration  calDispType=Number  calEnum={'False', 'True'}  calGain=1.0  calOffset=0.0  calMax=inf  calMin=-inf  calFormat='-1'  calUnit=''  calHelp=''  calAccess=1  calFunction=raptor_xcp_function(gcb)  calDispHeaders=off  calColHeaders={'Col1' 'Col2' 'Col3'}  calRowHeaders={'Row1' 'Row2' 'Row3'}
      settings: SourceProductName=Raptor
  raptor_fault_def : Raptor_lib/Faults/raptor_fault_def  faultName='IN_CAN2_500_Fault'  persist=on  sticky=off  emisRelated=off  permanent=off  singleTrip=off  clearMethod=Standard  xLimit=25  yLimit=50  calEnable=on  addDisable=off  calAccess=1  calFunction='System | FaultManager'
      settings: SourceProductName=Raptor
  raptor_fault_def1 : Raptor_lib/Faults/raptor_fault_def  faultName='IN_CAN2_501_Fault'  persist=on  sticky=off  emisRelated=off  permanent=off  singleTrip=off  clearMethod=Standard  xLimit=25  yLimit=50  calEnable=on  addDisable=off  calAccess=1  calFunction='System | FaultManager'
      settings: SourceProductName=Raptor
  raptor_fault_def10 : Raptor_lib/Faults/raptor_fault_def  faultName='IN_CAN2_510_Fault'  persist=on  sticky=off  emisRelated=off  permanent=off  singleTrip=off  clearMethod=Standard  xLimit=25  yLimit=50  calEnable=on  addDisable=off  calAccess=1  calFunction='System | FaultManager'
      settings: SourceProductName=Raptor
  raptor_fault_def11 : Raptor_lib/Faults/raptor_fault_def  faultName='IN_CAN2_511_Fault'  persist=on  sticky=off  emisRelated=off  permanent=off  singleTrip=off  clearMethod=Standard  xLimit=25  yLimit=50  calEnable=on  addDisable=off  calAccess=1  calFunction='System | FaultManager'
      settings: SourceProductName=Raptor
  raptor_fault_def12 : Raptor_lib/Faults/raptor_fault_def  faultName='IN_CAN2_512_Fault'  persist=on  sticky=off  emisRelated=off  permanent=off  singleTrip=off  clearMethod=Standard  xLimit=25  yLimit=50  calEnable=on  addDisable=off  calAccess=1  calFunction='System | FaultManager'
      settings: SourceProductName=Raptor
  raptor_fault_def13 : Raptor_lib/Faults/raptor_fault_def  faultName='IN_CAN2_513_Fault'  persist=on  sticky=off  emisRelated=off  permanent=off  singleTrip=off  clearMethod=Standard  xLimit=25  yLimit=50  calEnable=on  addDisable=off  calAccess=1  calFunction='System | FaultManager'
      settings: SourceProductName=Raptor
  raptor_fault_def14 : Raptor_lib/Faults/raptor_fault_def  faultName='IN_CAN2_513_Fault'  persist=on  sticky=off  emisRelated=off  permanent=off  singleTrip=off  clearMethod=Standard  xLimit=25  yLimit=50  calEnable=on  addDisable=off  calAccess=1  calFunction='System | FaultManager'
      settings: SourceProductName=Raptor
  raptor_fault_def15 : Raptor_lib/Faults/raptor_fault_def  faultName='IN_CAN2_515_Fault'  persist=on  sticky=off  emisRelated=off  permanent=off  singleTrip=off  clearMethod=Standard  xLimit=25  yLimit=50  calEnable=on  addDisable=off  calAccess=1  calFunction='System | FaultManager'
      settings: SourceProductName=Raptor
  raptor_fault_def16 : Raptor_lib/Faults/raptor_fault_def  faultName='IN_CAN2_516_Fault'  persist=on  sticky=off  emisRelated=off  permanent=off  singleTrip=off  clearMethod=Standard  xLimit=25  yLimit=50  calEnable=on  addDisable=off  calAccess=1  calFunction='System | FaultManager'
      settings: SourceProductName=Raptor
  raptor_fault_def17 : Raptor_lib/Faults/raptor_fault_def  faultName='IN_CAN2_517_Fault'  persist=on  sticky=off  emisRelated=off  permanent=off  singleTrip=off  clearMethod=Standard  xLimit=25  yLimit=50  calEnable=on  addDisable=off  calAccess=1  calFunction='System | FaultManager'
      settings: SourceProductName=Raptor
  raptor_fault_def18 : Raptor_lib/Faults/raptor_fault_def  faultName='IN_CAN2_526_Fault'  persist=on  sticky=off  emisRelated=off  permanent=off  singleTrip=off  clearMethod=Standard  xLimit=25  yLimit=50  calEnable=on  addDisable=off  calAccess=1  calFunction='System | FaultManager'
      settings: SourceProductName=Raptor
  raptor_fault_def19 : Raptor_lib/Faults/raptor_fault_def  faultName='IN_CAN2_527_Fault'  persist=on  sticky=off  emisRelated=off  permanent=off  singleTrip=off  clearMethod=Standard  xLimit=25  yLimit=50  calEnable=on  addDisable=off  calAccess=1  calFunction='System | FaultManager'
      settings: SourceProductName=Raptor
  raptor_fault_def2 : Raptor_lib/Faults/raptor_fault_def  faultName='IN_CAN2_502_Fault'  persist=on  sticky=off  emisRelated=off  permanent=off  singleTrip=off  clearMethod=Standard  xLimit=25  yLimit=50  calEnable=on  addDisable=off  calAccess=1  calFunction='System | FaultManager'
      settings: SourceProductName=Raptor
  raptor_fault_def20 : Raptor_lib/Faults/raptor_fault_def  faultName='IN_CAN2_528_Fault'  persist=on  sticky=off  emisRelated=off  permanent=off  singleTrip=off  clearMethod=Standard  xLimit=25  yLimit=50  calEnable=on  addDisable=off  calAccess=1  calFunction='System | FaultManager'
      settings: SourceProductName=Raptor
  raptor_fault_def21 : Raptor_lib/Faults/raptor_fault_def  faultName='IN_CAN2_529_Fault'  persist=on  sticky=off  emisRelated=off  permanent=off  singleTrip=off  clearMethod=Standard  xLimit=25  yLimit=50  calEnable=on  addDisable=off  calAccess=1  calFunction='System | FaultManager'
      settings: SourceProductName=Raptor
  raptor_fault_def22 : Raptor_lib/Faults/raptor_fault_def  faultName='IN_CAN2_530_Fault'  persist=on  sticky=off  emisRelated=off  permanent=off  singleTrip=off  clearMethod=Standard  xLimit=25  yLimit=50  calEnable=on  addDisable=off  calAccess=1  calFunction='System | FaultManager'
      settings: SourceProductName=Raptor
  raptor_fault_def23 : Raptor_lib/Faults/raptor_fault_def  faultName='IN_CAN2_530_Fault'  persist=on  sticky=off  emisRelated=off  permanent=off  singleTrip=off  clearMethod=Standard  xLimit=25  yLimit=50  calEnable=on  addDisable=off  calAccess=1  calFunction='System | FaultManager'
      settings: SourceProductName=Raptor
  raptor_fault_def24 : Raptor_lib/Faults/raptor_fault_def  faultName='IN_CAN2_518_Fault'  persist=on  sticky=off  emisRelated=off  permanent=off  singleTrip=off  clearMethod=Standard  xLimit=25  yLimit=50  calEnable=on  addDisable=off  calAccess=1  calFunction='System | FaultManager'
      settings: SourceProductName=Raptor
  raptor_fault_def25 : Raptor_lib/Faults/raptor_fault_def  faultName='IN_CAN2_519_Fault'  persist=on  sticky=off  emisRelated=off  permanent=off  singleTrip=off  clearMethod=Standard  xLimit=25  yLimit=50  calEnable=on  addDisable=off  calAccess=1  calFunction='System | FaultManager'
      settings: SourceProductName=Raptor
  raptor_fault_def26 : Raptor_lib/Faults/raptor_fault_def  faultName='IN_CAN2_520_Fault'  persist=on  sticky=off  emisRelated=off  permanent=off  singleTrip=off  clearMethod=Standard  xLimit=25  yLimit=50  calEnable=on  addDisable=off  calAccess=1  calFunction='System | FaultManager'
      settings: SourceProductName=Raptor
  raptor_fault_def27 : Raptor_lib/Faults/raptor_fault_def  faultName='IN_CAN2_521_Fault'  persist=on  sticky=off  emisRelated=off  permanent=off  singleTrip=off  clearMethod=Standard  xLimit=25  yLimit=50  calEnable=on  addDisable=off  calAccess=1  calFunction='System | FaultManager'
      settings: SourceProductName=Raptor
  raptor_fault_def28 : Raptor_lib/Faults/raptor_fault_def  faultName='IN_CAN2_522_Fault'  persist=on  sticky=off  emisRelated=off  permanent=off  singleTrip=off  clearMethod=Standard  xLimit=25  yLimit=50  calEnable=on  addDisable=off  calAccess=1  calFunction='System | FaultManager'
      settings: SourceProductName=Raptor
  raptor_fault_def29 : Raptor_lib/Faults/raptor_fault_def  faultName='IN_CAN2_523_Fault'  persist=on  sticky=off  emisRelated=off  permanent=off  singleTrip=off  clearMethod=Standard  xLimit=25  yLimit=50  calEnable=on  addDisable=off  calAccess=1  calFunction='System | FaultManager'
      settings: SourceProductName=Raptor
  raptor_fault_def3 : Raptor_lib/Faults/raptor_fault_def  faultName='IN_CAN2_503_Fault'  persist=on  sticky=off  emisRelated=off  permanent=off  singleTrip=off  clearMethod=Standard  xLimit=25  yLimit=50  calEnable=on  addDisable=off  calAccess=1  calFunction='System | FaultManager'
      settings: SourceProductName=Raptor
  raptor_fault_def30 : Raptor_lib/Faults/raptor_fault_def  faultName='IN_CAN2_524_Fault'  persist=on  sticky=off  emisRelated=off  permanent=off  singleTrip=off  clearMethod=Standard  xLimit=25  yLimit=50  calEnable=on  addDisable=off  calAccess=1  calFunction='System | FaultManager'
      settings: SourceProductName=Raptor
  raptor_fault_def31 : Raptor_lib/Faults/raptor_fault_def  faultName='IN_CAN2_525_Fault'  persist=on  sticky=off  emisRelated=off  permanent=off  singleTrip=off  clearMethod=Standard  xLimit=25  yLimit=50  calEnable=on  addDisable=off  calAccess=1  calFunction='System | FaultManager'
      settings: SourceProductName=Raptor
  raptor_fault_def33 : Raptor_lib/Faults/raptor_fault_def  faultName='IN_CAN2_532_Fault'  persist=on  sticky=off  emisRelated=off  permanent=off  singleTrip=off  clearMethod=Standard  xLimit=25  yLimit=50  calEnable=on  addDisable=off  calAccess=1  calFunction='System | FaultManager'
      settings: SourceProductName=Raptor
  raptor_fault_def34 : Raptor_lib/Faults/raptor_fault_def  faultName='IN_CAN2_541_Fault'  persist=on  sticky=off  emisRelated=off  permanent=off  singleTrip=off  clearMethod=Standard  xLimit=25  yLimit=50  calEnable=on  addDisable=off  calAccess=1  calFunction='System | FaultManager'
      settings: SourceProductName=Raptor
  raptor_fault_def35 : Raptor_lib/Faults/raptor_fault_def  faultName='IN_CAN2_542_Fault'  persist=on  sticky=off  emisRelated=off  permanent=off  singleTrip=off  clearMethod=Standard  xLimit=25  yLimit=50  calEnable=on  addDisable=off  calAccess=1  calFunction='System | FaultManager'
      settings: SourceProductName=Raptor
  raptor_fault_def36 : Raptor_lib/Faults/raptor_fault_def  faultName='IN_CAN2_543_Fault'  persist=on  sticky=off  emisRelated=off  permanent=off  singleTrip=off  clearMethod=Standard  xLimit=25  yLimit=50  calEnable=on  addDisable=off  calAccess=1  calFunction='System | FaultManager'
      settings: SourceProductName=Raptor
  raptor_fault_def37 : Raptor_lib/Faults/raptor_fault_def  faultName='IN_CAN2_544_Fault'  persist=on  sticky=off  emisRelated=off  permanent=off  singleTrip=off  clearMethod=Standard  xLimit=25  yLimit=50  calEnable=on  addDisable=off  calAccess=1  calFunction='System | FaultManager'
      settings: SourceProductName=Raptor
  raptor_fault_def38 : Raptor_lib/Faults/raptor_fault_def  faultName='IN_CAN2_545_Fault'  persist=on  sticky=off  emisRelated=off  permanent=off  singleTrip=off  clearMethod=Standard  xLimit=25  yLimit=50  calEnable=on  addDisable=off  calAccess=1  calFunction='System | FaultManager'
      settings: SourceProductName=Raptor
  raptor_fault_def39 : Raptor_lib/Faults/raptor_fault_def  faultName='IN_CAN2_546_Fault'  persist=on  sticky=off  emisRelated=off  permanent=off  singleTrip=off  clearMethod=Standard  xLimit=25  yLimit=50  calEnable=on  addDisable=off  calAccess=1  calFunction='System | FaultManager'
      settings: SourceProductName=Raptor
  raptor_fault_def4 : Raptor_lib/Faults/raptor_fault_def  faultName='IN_CAN2_504_Fault'  persist=on  sticky=off  emisRelated=off  permanent=off  singleTrip=off  clearMethod=Standard  xLimit=25  yLimit=50  calEnable=on  addDisable=off  calAccess=1  calFunction='System | FaultManager'
      settings: SourceProductName=Raptor
  raptor_fault_def40 : Raptor_lib/Faults/raptor_fault_def  faultName='IN_CAN2_547_Fault'  persist=on  sticky=off  emisRelated=off  permanent=off  singleTrip=off  clearMethod=Standard  xLimit=25  yLimit=50  calEnable=on  addDisable=off  calAccess=1  calFunction='System | FaultManager'
      settings: SourceProductName=Raptor
  raptor_fault_def41 : Raptor_lib/Faults/raptor_fault_def  faultName='IN_CAN2_548_Fault'  persist=on  sticky=off  emisRelated=off  permanent=off  singleTrip=off  clearMethod=Standard  xLimit=25  yLimit=50  calEnable=on  addDisable=off  calAccess=1  calFunction='System | FaultManager'
      settings: SourceProductName=Raptor
  raptor_fault_def42 : Raptor_lib/Faults/raptor_fault_def  faultName='IN_CAN2_557_Fault'  persist=on  sticky=off  emisRelated=off  permanent=off  singleTrip=off  clearMethod=Standard  xLimit=25  yLimit=50  calEnable=on  addDisable=off  calAccess=1  calFunction='System | FaultManager'
      settings: SourceProductName=Raptor
  raptor_fault_def43 : Raptor_lib/Faults/raptor_fault_def  faultName='IN_CAN2_558_Fault'  persist=on  sticky=off  emisRelated=off  permanent=off  singleTrip=off  clearMethod=Standard  xLimit=25  yLimit=50  calEnable=on  addDisable=off  calAccess=1  calFunction='System | FaultManager'
      settings: SourceProductName=Raptor
  raptor_fault_def44 : Raptor_lib/Faults/raptor_fault_def  faultName='IN_CAN2_533_Fault'  persist=on  sticky=off  emisRelated=off  permanent=off  singleTrip=off  clearMethod=Standard  xLimit=25  yLimit=50  calEnable=on  addDisable=off  calAccess=1  calFunction='System | FaultManager'
      settings: SourceProductName=Raptor
  raptor_fault_def45 : Raptor_lib/Faults/raptor_fault_def  faultName='IN_CAN2_559_Fault'  persist=on  sticky=off  emisRelated=off  permanent=off  singleTrip=off  clearMethod=Standard  xLimit=25  yLimit=50  calEnable=on  addDisable=off  calAccess=1  calFunction='System | FaultManager'
      settings: SourceProductName=Raptor
  raptor_fault_def46 : Raptor_lib/Faults/raptor_fault_def  faultName='IN_CAN2_560_Fault'  persist=on  sticky=off  emisRelated=off  permanent=off  singleTrip=off  clearMethod=Standard  xLimit=25  yLimit=50  calEnable=on  addDisable=off  calAccess=1  calFunction='System | FaultManager'
      settings: SourceProductName=Raptor
  raptor_fault_def47 : Raptor_lib/Faults/raptor_fault_def  faultName='IN_CAN2_561_Fault'  persist=on  sticky=off  emisRelated=off  permanent=off  singleTrip=off  clearMethod=Standard  xLimit=25  yLimit=50  calEnable=on  addDisable=off  calAccess=1  calFunction='System | FaultManager'
      settings: SourceProductName=Raptor
  raptor_fault_def48 : Raptor_lib/Faults/raptor_fault_def  faultName='IN_CAN2_562_Fault'  persist=on  sticky=off  emisRelated=off  permanent=off  singleTrip=off  clearMethod=Standard  xLimit=25  yLimit=50  calEnable=on  addDisable=off  calAccess=1  calFunction='System | FaultManager'
      settings: SourceProductName=Raptor
  raptor_fault_def49 : Raptor_lib/Faults/raptor_fault_def  faultName='IN_CAN2_549_Fault'  persist=on  sticky=off  emisRelated=off  permanent=off  singleTrip=off  clearMethod=Standard  xLimit=25  yLimit=50  calEnable=on  addDisable=off  calAccess=1  calFunction='System | FaultManager'
      settings: SourceProductName=Raptor
  raptor_fault_def5 : Raptor_lib/Faults/raptor_fault_def  faultName='IN_CAN2_505_Fault'  persist=on  sticky=off  emisRelated=off  permanent=off  singleTrip=off  clearMethod=Standard  xLimit=25  yLimit=50  calEnable=on  addDisable=off  calAccess=1  calFunction='System | FaultManager'
      settings: SourceProductName=Raptor
  raptor_fault_def50 : Raptor_lib/Faults/raptor_fault_def  faultName='IN_CAN2_550_Fault'  persist=on  sticky=off  emisRelated=off  permanent=off  singleTrip=off  clearMethod=Standard  xLimit=25  yLimit=50  calEnable=on  addDisable=off  calAccess=1  calFunction='System | FaultManager'
      settings: SourceProductName=Raptor
  raptor_fault_def51 : Raptor_lib/Faults/raptor_fault_def  faultName='IN_CAN2_551_Fault'  persist=on  sticky=off  emisRelated=off  permanent=off  singleTrip=off  clearMethod=Standard  xLimit=25  yLimit=50  calEnable=on  addDisable=off  calAccess=1  calFunction='System | FaultManager'
      settings: SourceProductName=Raptor
  raptor_fault_def52 : Raptor_lib/Faults/raptor_fault_def  faultName='IN_CAN2_552_Fault'  persist=on  sticky=off  emisRelated=off  permanent=off  singleTrip=off  clearMethod=Standard  xLimit=25  yLimit=50  calEnable=on  addDisable=off  calAccess=1  calFunction='System | FaultManager'
      settings: SourceProductName=Raptor
  raptor_fault_def53 : Raptor_lib/Faults/raptor_fault_def  faultName='IN_CAN2_553_Fault'  persist=on  sticky=off  emisRelated=off  permanent=off  singleTrip=off  clearMethod=Standard  xLimit=25  yLimit=50  calEnable=on  addDisable=off  calAccess=1  calFunction='System | FaultManager'
      settings: SourceProductName=Raptor
  raptor_fault_def54 : Raptor_lib/Faults/raptor_fault_def  faultName='IN_CAN2_554_Fault'  persist=on  sticky=off  emisRelated=off  permanent=off  singleTrip=off  clearMethod=Standard  xLimit=25  yLimit=50  calEnable=on  addDisable=off  calAccess=1  calFunction='System | FaultManager'
      settings: SourceProductName=Raptor
  raptor_fault_def55 : Raptor_lib/Faults/raptor_fault_def  faultName='IN_CAN2_534_Fault'  persist=on  sticky=off  emisRelated=off  permanent=off  singleTrip=off  clearMethod=Standard  xLimit=25  yLimit=50  calEnable=on  addDisable=off  calAccess=1  calFunction='System | FaultManager'
      settings: SourceProductName=Raptor
  raptor_fault_def56 : Raptor_lib/Faults/raptor_fault_def  faultName='IN_CAN2_555_Fault'  persist=on  sticky=off  emisRelated=off  permanent=off  singleTrip=off  clearMethod=Standard  xLimit=25  yLimit=50  calEnable=on  addDisable=off  calAccess=1  calFunction='System | FaultManager'
      settings: SourceProductName=Raptor
  raptor_fault_def57 : Raptor_lib/Faults/raptor_fault_def  faultName='IN_CAN2_556_Fault'  persist=on  sticky=off  emisRelated=off  permanent=off  singleTrip=off  clearMethod=Standard  xLimit=25  yLimit=50  calEnable=on  addDisable=off  calAccess=1  calFunction='System | FaultManager'
      settings: SourceProductName=Raptor
  raptor_fault_def58 : Raptor_lib/Faults/raptor_fault_def  faultName='IN_CAN2_535_Fault'  persist=on  sticky=off  emisRelated=off  permanent=off  singleTrip=off  clearMethod=Standard  xLimit=25  yLimit=50  calEnable=on  addDisable=off  calAccess=1  calFunction='System | FaultManager'
      settings: SourceProductName=Raptor
  raptor_fault_def59 : Raptor_lib/Faults/raptor_fault_def  faultName='IN_CAN2_536_Fault'  persist=on  sticky=off  emisRelated=off  permanent=off  singleTrip=off  clearMethod=Standard  xLimit=25  yLimit=50  calEnable=on  addDisable=off  calAccess=1  calFunction='System | FaultManager'
      settings: SourceProductName=Raptor
  raptor_fault_def6 : Raptor_lib/Faults/raptor_fault_def  faultName='IN_CAN2_506_Fault'  persist=on  sticky=off  emisRelated=off  permanent=off  singleTrip=off  clearMethod=Standard  xLimit=25  yLimit=50  calEnable=on  addDisable=off  calAccess=1  calFunction='System | FaultManager'
      settings: SourceProductName=Raptor
  raptor_fault_def60 : Raptor_lib/Faults/raptor_fault_def  faultName='IN_CAN2_537_Fault'  persist=on  sticky=off  emisRelated=off  permanent=off  singleTrip=off  clearMethod=Standard  xLimit=25  yLimit=50  calEnable=on  addDisable=off  calAccess=1  calFunction='System | FaultManager'
      settings: SourceProductName=Raptor
  raptor_fault_def61 : Raptor_lib/Faults/raptor_fault_def  faultName='IN_CAN2_538_Fault'  persist=on  sticky=off  emisRelated=off  permanent=off  singleTrip=off  clearMethod=Standard  xLimit=25  yLimit=50  calEnable=on  addDisable=off  calAccess=1  calFunction='System | FaultManager'
      settings: SourceProductName=Raptor
  raptor_fault_def62 : Raptor_lib/Faults/raptor_fault_def  faultName='IN_CAN2_539_Fault'  persist=on  sticky=off  emisRelated=off  permanent=off  singleTrip=off  clearMethod=Standard  xLimit=25  yLimit=50  calEnable=on  addDisable=off  calAccess=1  calFunction='System | FaultManager'
      settings: SourceProductName=Raptor
  raptor_fault_def63 : Raptor_lib/Faults/raptor_fault_def  faultName='IN_CAN2_540_Fault'  persist=on  sticky=off  emisRelated=off  permanent=off  singleTrip=off  clearMethod=Standard  xLimit=25  yLimit=50  calEnable=on  addDisable=off  calAccess=1  calFunction='System | FaultManager'
      settings: SourceProductName=Raptor
  raptor_fault_def7 : Raptor_lib/Faults/raptor_fault_def  faultName='IN_CAN2_507_Fault'  persist=on  sticky=off  emisRelated=off  permanent=off  singleTrip=off  clearMethod=Standard  xLimit=25  yLimit=50  calEnable=on  addDisable=off  calAccess=1  calFunction='System | FaultManager'
      settings: SourceProductName=Raptor
  raptor_fault_def8 : Raptor_lib/Faults/raptor_fault_def  faultName='IN_CAN2_508_Fault'  persist=on  sticky=off  emisRelated=off  permanent=off  singleTrip=off  clearMethod=Standard  xLimit=25  yLimit=50  calEnable=on  addDisable=off  calAccess=1  calFunction='System | FaultManager'
      settings: SourceProductName=Raptor
  raptor_fault_def9 : Raptor_lib/Faults/raptor_fault_def  faultName='IN_CAN2_509_Fault'  persist=on  sticky=off  emisRelated=off  permanent=off  singleTrip=off  clearMethod=Standard  xLimit=25  yLimit=50  calEnable=on  addDisable=off  calAccess=1  calFunction='System | FaultManager'
      settings: SourceProductName=Raptor
  Out1 : Outport
  wires:
  Mux/1 -> CANTimeoutCheck/1
  EnumeratedOverMeas1/1 -> Mux1/2  "IN_CAN1_302_Status_en"
  raptor_adjustment1/1 -> RollingCounterCheck/Enable, RollingCounterCheck/2
  [IO_CAN2_502_Age] -> Mux2/3
  raptor_adjustment/1 -> CANTimeoutCheck/2
  CANTimeoutCheck/1 -> Demux/1
  [IO_CAN2_502_cnt] -> Mux/3
  [IO_CAN2_501_Age] -> Mux2/2
  Demux/2 -> EnumeratedOverMeas1/1
  Demux/1 -> EnumeratedOverMeas/1
  [IO_CAN2_500_Age] -> Mux2/1
  [IO_CAN2_501_cnt] -> Mux/2
  EnumeratedOverMeas2/1 -> Mux1/3  "IN_CAN1_303_Staus_en"
  EnumeratedOverMeas4/1 -> Mux1/4  "IN_CAN1_305_Status_en"
  Mux1/1 -> Equal/1
  RollingCounterCheck/1 -> Logical Operator/1
  Demux1/1 -> raptor_fault_def/1, [IN_CAN2_500_Fault]
  Demux/3 -> EnumeratedOverMeas2/1
  Enumerated Constant/1 -> Equal/2
  [IO_CAN2_503_cnt] -> Mux/4
  Logical Operator/1 -> Demux1/1
  [IO_CAN2_503_Age] -> Mux2/4
  Equal/1 -> Logical Operator/2
  [IO_CAN2_500_cnt] -> Mux/1
  Demux/4 -> EnumeratedOverMeas4/1
  EnumeratedOverMeas/1 -> Mux1/1  "IN_CAN1_301_Status_en"
  Mux2/1 -> RollingCounterCheck/1
  [IO_CAN2_504_cnt] -> Mux/5
  [IO_CAN2_505_cnt] -> Mux/6
  [IO_CAN2_506_cnt] -> Mux/7
  [IO_CAN2_507_cnt] -> Mux/8
  [IO_CAN2_508_cnt] -> Mux/9
  [IO_CAN2_509_cnt] -> Mux/10
  [IO_CAN2_510_cnt] -> Mux/11
  [IO_CAN2_511_cnt] -> Mux/12
  [IO_CAN2_512_cnt] -> Mux/13
  [IO_CAN2_513_cnt] -> Mux/14
  [IO_CAN2_514_cnt] -> Mux/15
  [IO_CAN2_515_cnt] -> Mux/16
  [IO_CAN2_516_cnt] -> Mux/17
  [IO_CAN2_517_cnt] -> Mux/18
  [IO_CAN2_518_cnt] -> Mux/19
  [IO_CAN2_519_cnt] -> Mux/20
  [IO_CAN2_520_cnt] -> Mux/21
  [IO_CAN2_521_cnt] -> Mux/22
  [IO_CAN2_522_cnt] -> Mux/23
  [IO_CAN2_523_cnt] -> Mux/24
  [IO_CAN2_524_cnt] -> Mux/25
  [IO_CAN2_525_cnt] -> Mux/26
  [IO_CAN2_526_cnt] -> Mux/27
  [IO_CAN2_527_cnt] -> Mux/28
  [IO_CAN2_528_cnt] -> Mux/29
  [IO_CAN2_529_cnt] -> Mux/30
  [IO_CAN2_530_cnt] -> Mux/31
  [IO_CAN2_531_cnt] -> Mux/32
  [IO_CAN2_532_cnt] -> Mux/33
  [IO_CAN2_533_cnt] -> Mux/34
  [IO_CAN2_534_cnt] -> Mux/35
  [IO_CAN2_535_cnt] -> Mux/36
  [IO_CAN2_536_cnt] -> Mux/37
  [IO_CAN2_537_cnt] -> Mux/38
  [IO_CAN2_538_cnt] -> Mux/39
  [IO_CAN2_539_cnt] -> Mux/40
  [IO_CAN2_540_cnt] -> Mux/41
  [IO_CAN2_541_cnt] -> Mux/42
  [IO_CAN2_542_cnt] -> Mux/43
  [IO_CAN2_543_cnt] -> Mux/44
  [IO_CAN2_544_cnt] -> Mux/45
  [IO_CAN2_545_cnt] -> Mux/46
  [IO_CAN1_303_Age] -> Mux/47
  [IO_CAN1_305_Age] -> Mux/48
  [IO_CAN1_301_Age] -> Mux/49
  [IO_CAN1_302_Age] -> Mux/50
  [IO_CAN1_303_Age] -> Mux/51
  [IO_CAN1_305_Age] -> Mux/52
  [IO_CAN1_301_Age] -> Mux/53
  [IO_CAN1_302_Age] -> Mux/54
  [IO_CAN1_303_Age] -> Mux/55
  [IO_CAN1_305_Age] -> Mux/56
  [IO_CAN1_301_Age] -> Mux/57
  [IO_CAN1_302_Age] -> Mux/58
  [IO_CAN1_303_Age] -> Mux/59
  [IO_CAN1_305_Age] -> Mux/60
  [IO_CAN1_301_Age] -> Mux/61
  [IO_CAN1_302_Age] -> Mux/62
  [IO_CAN1_303_Age] -> Mux/63
  EnumeratedOverMeas3/1 -> Mux1/5  "IN_CAN1_301_Status_en"
  EnumeratedOverMeas5/1 -> Mux1/6  "IN_CAN1_302_Status_en"
  EnumeratedOverMeas6/1 -> Mux1/7  "IN_CAN1_303_Staus_en"
  EnumeratedOverMeas7/1 -> Mux1/8  "IN_CAN1_305_Status_en"
  Demux/5 -> EnumeratedOverMeas3/1
  Demux/6 -> EnumeratedOverMeas5/1
  Demux/7 -> EnumeratedOverMeas6/1
  Demux/8 -> EnumeratedOverMeas7/1
  Demux/16 -> EnumeratedOverMeas15/1
  Demux/15 -> EnumeratedOverMeas14/1
  Demux/14 -> EnumeratedOverMeas13/1
  Demux/13 -> EnumeratedOverMeas11/1
  EnumeratedOverMeas15/1 -> Mux1/16  "IN_CAN1_305_Status_en"
  EnumeratedOverMeas14/1 -> Mux1/15  "IN_CAN1_303_Staus_en"
  EnumeratedOverMeas13/1 -> Mux1/14  "IN_CAN1_302_Status_en"
  EnumeratedOverMeas11/1 -> Mux1/13  "IN_CAN1_301_Status_en"
  EnumeratedOverMeas8/1 -> Mux1/9  "IN_CAN1_301_Status_en"
  Demux/12 -> EnumeratedOverMeas12/1
  Demux/11 -> EnumeratedOverMeas10/1
  EnumeratedOverMeas12/1 -> Mux1/12  "IN_CAN1_305_Status_en"
  EnumeratedOverMeas10/1 -> Mux1/11  "IN_CAN1_303_Staus_en"
  Demux/9 -> EnumeratedOverMeas8/1
  Demux/10 -> EnumeratedOverMeas9/1
  EnumeratedOverMeas9/1 -> Mux1/10  "IN_CAN1_302_Status_en"
  EnumeratedOverMeas31/1 -> Mux1/26  "IN_CAN1_302_Status_en"
  Demux/26 -> EnumeratedOverMeas31/1
  Demux/25 -> EnumeratedOverMeas30/1
  EnumeratedOverMeas18/1 -> Mux1/27  "IN_CAN1_303_Staus_en"
  EnumeratedOverMeas20/1 -> Mux1/28  "IN_CAN1_305_Status_en"
  Demux/27 -> EnumeratedOverMeas18/1
  Demux/28 -> EnumeratedOverMeas20/1
  EnumeratedOverMeas30/1 -> Mux1/25  "IN_CAN1_301_Status_en"
  EnumeratedOverMeas19/1 -> Mux1/29  "IN_CAN1_301_Status_en"
  EnumeratedOverMeas21/1 -> Mux1/30  "IN_CAN1_302_Status_en"
  EnumeratedOverMeas22/1 -> Mux1/31  "IN_CAN1_303_Staus_en"
  EnumeratedOverMeas23/1 -> Mux1/32  "IN_CAN1_305_Status_en"
  Demux/29 -> EnumeratedOverMeas19/1
  Demux/30 -> EnumeratedOverMeas21/1
  Demux/31 -> EnumeratedOverMeas22/1
  Demux/32 -> EnumeratedOverMeas23/1
  Demux/24 -> EnumeratedOverMeas29/1
  Demux/23 -> EnumeratedOverMeas28/1
  Demux/22 -> EnumeratedOverMeas27/1
  Demux/21 -> EnumeratedOverMeas25/1
  EnumeratedOverMeas29/1 -> Mux1/24  "IN_CAN1_305_Status_en"
  EnumeratedOverMeas28/1 -> Mux1/23  "IN_CAN1_303_Staus_en"
  EnumeratedOverMeas27/1 -> Mux1/22  "IN_CAN1_302_Status_en"
  EnumeratedOverMeas25/1 -> Mux1/21  "IN_CAN1_301_Status_en"
  EnumeratedOverMeas16/1 -> Mux1/17  "IN_CAN1_301_Status_en"
  Demux/20 -> EnumeratedOverMeas26/1
  Demux/19 -> EnumeratedOverMeas24/1
  EnumeratedOverMeas26/1 -> Mux1/20  "IN_CAN1_305_Status_en"
  EnumeratedOverMeas24/1 -> Mux1/19  "IN_CAN1_303_Staus_en"
  Demux/17 -> EnumeratedOverMeas16/1
  Demux/18 -> EnumeratedOverMeas17/1
  EnumeratedOverMeas17/1 -> Mux1/18  "IN_CAN1_302_Status_en"
  EnumeratedOverMeas41/1 -> Mux1/50  "IN_CAN1_302_Status_en"
  Demux/50 -> EnumeratedOverMeas41/1
  Demux/49 -> EnumeratedOverMeas40/1
  EnumeratedOverMeas49/1 -> Mux1/51  "IN_CAN1_303_Staus_en"
  EnumeratedOverMeas51/1 -> Mux1/52  "IN_CAN1_305_Status_en"
  Demux/51 -> EnumeratedOverMeas49/1
  Demux/52 -> EnumeratedOverMeas51/1
  EnumeratedOverMeas40/1 -> Mux1/49  "IN_CAN1_301_Status_en"
  EnumeratedOverMeas50/1 -> Mux1/53  "IN_CAN1_301_Status_en"
  EnumeratedOverMeas52/1 -> Mux1/54  "IN_CAN1_302_Status_en"
  EnumeratedOverMeas53/1 -> Mux1/55  "IN_CAN1_303_Staus_en"
  EnumeratedOverMeas54/1 -> Mux1/56  "IN_CAN1_305_Status_en"
  Demux/53 -> EnumeratedOverMeas50/1
  Demux/54 -> EnumeratedOverMeas52/1
  Demux/55 -> EnumeratedOverMeas53/1
  Demux/56 -> EnumeratedOverMeas54/1
  Demux/63 -> EnumeratedOverMeas47/1
  Demux/62 -> EnumeratedOverMeas46/1
  Demux/61 -> EnumeratedOverMeas43/1
  EnumeratedOverMeas47/1 -> Mux1/63  "IN_CAN1_303_Staus_en"
  EnumeratedOverMeas46/1 -> Mux1/62  "IN_CAN1_302_Status_en"
  EnumeratedOverMeas43/1 -> Mux1/61  "IN_CAN1_301_Status_en"
  EnumeratedOverMeas56/1 -> Mux1/57  "IN_CAN1_301_Status_en"
  Demux/60 -> EnumeratedOverMeas45/1
  Demux/59 -> EnumeratedOverMeas42/1
  EnumeratedOverMeas45/1 -> Mux1/60  "IN_CAN1_305_Status_en"
  EnumeratedOverMeas42/1 -> Mux1/59  "IN_CAN1_303_Staus_en"
  Demux/57 -> EnumeratedOverMeas56/1
  Demux/58 -> EnumeratedOverMeas57/1
  EnumeratedOverMeas57/1 -> Mux1/58  "IN_CAN1_302_Status_en"
  EnumeratedOverMeas63/1 -> Mux1/42  "IN_CAN1_302_Status_en"
  Demux/42 -> EnumeratedOverMeas63/1
  Demux/41 -> EnumeratedOverMeas62/1
  EnumeratedOverMeas34/1 -> Mux1/43  "IN_CAN1_303_Staus_en"
  EnumeratedOverMeas36/1 -> Mux1/44  "IN_CAN1_305_Status_en"
  Demux/43 -> EnumeratedOverMeas34/1
  Demux/44 -> EnumeratedOverMeas36/1
  EnumeratedOverMeas62/1 -> Mux1/41  "IN_CAN1_301_Status_en"
  EnumeratedOverMeas35/1 -> Mux1/45  "IN_CAN1_301_Status_en"
  EnumeratedOverMeas37/1 -> Mux1/46  "IN_CAN1_302_Status_en"
  EnumeratedOverMeas38/1 -> Mux1/47  "IN_CAN1_303_Staus_en"
  EnumeratedOverMeas39/1 -> Mux1/48  "IN_CAN1_305_Status_en"
  Demux/45 -> EnumeratedOverMeas35/1
  Demux/46 -> EnumeratedOverMeas37/1
  Demux/47 -> EnumeratedOverMeas38/1
  Demux/48 -> EnumeratedOverMeas39/1
  Demux/40 -> EnumeratedOverMeas61/1
  Demux/39 -> EnumeratedOverMeas60/1
  Demux/38 -> EnumeratedOverMeas59/1
  Demux/37 -> EnumeratedOverMeas55/1
  EnumeratedOverMeas61/1 -> Mux1/40  "IN_CAN1_305_Status_en"
  EnumeratedOverMeas60/1 -> Mux1/39  "IN_CAN1_303_Staus_en"
  EnumeratedOverMeas59/1 -> Mux1/38  "IN_CAN1_302_Status_en"
  EnumeratedOverMeas55/1 -> Mux1/37  "IN_CAN1_301_Status_en"
  EnumeratedOverMeas32/1 -> Mux1/33  "IN_CAN1_301_Status_en"
  Demux/36 -> EnumeratedOverMeas58/1
  Demux/35 -> EnumeratedOverMeas44/1
  EnumeratedOverMeas58/1 -> Mux1/36  "IN_CAN1_305_Status_en"
  EnumeratedOverMeas44/1 -> Mux1/35  "IN_CAN1_303_Staus_en"
  Demux/33 -> EnumeratedOverMeas32/1
  Demux/34 -> EnumeratedOverMeas33/1
  EnumeratedOverMeas33/1 -> Mux1/34  "IN_CAN1_302_Status_en"
  [IO_CAN2_507_Age] -> Mux2/8
  [IO_CAN2_505_Age] -> Mux2/6
  [IO_CAN2_506_Age] -> Mux2/7
  [IO_CAN2_514_Age] -> Mux2/15
  [IO_CAN2_513_Age] -> Mux2/14
  [IO_CAN2_512_Age] -> Mux2/13
  [IO_CAN2_515_Age] -> Mux2/16
  [IO_CAN2_511_Age] -> Mux2/12
  [IO_CAN2_508_Age] -> Mux2/9
  [IO_CAN2_509_Age] -> Mux2/10
  [IO_CAN2_510_Age] -> Mux2/11
  [IO_CAN2_526_Age] -> Mux2/27
  [IO_CAN2_525_Age] -> Mux2/26
  [IO_CAN2_524_Age] -> Mux2/25
  [IO_CAN2_527_Age] -> Mux2/28
  [IO_CAN2_531_Age] -> Mux2/32
  [IO_CAN2_528_Age] -> Mux2/29
  [IO_CAN2_529_Age] -> Mux2/30
  [IO_CAN2_530_Age] -> Mux2/31
  [IO_CAN2_522_Age] -> Mux2/23
  [IO_CAN2_521_Age] -> Mux2/22
  [IO_CAN2_520_Age] -> Mux2/21
  [IO_CAN2_523_Age] -> Mux2/24
  [IO_CAN2_519_Age] -> Mux2/20
  [IO_CAN2_516_Age] -> Mux2/17
  [IO_CAN2_517_Age] -> Mux2/18
  [IO_CAN2_518_Age] -> Mux2/19
  [IO_CAN1_303_cnt] -> Mux2/51
  [IO_CAN1_302_cnt] -> Mux2/50
  [IO_CAN1_301_cnt] -> Mux2/49
  [IO_CAN1_305_cnt] -> Mux2/52
  [IO_CAN1_305_cnt] -> Mux2/56
  [IO_CAN1_301_cnt] -> Mux2/53
  [IO_CAN1_302_cnt] -> Mux2/54
  [IO_CAN1_303_cnt] -> Mux2/55
  [IO_CAN1_303_cnt] -> Mux2/63
  [IO_CAN1_302_cnt] -> Mux2/62
  [IO_CAN1_301_cnt] -> Mux2/61
  [IO_CAN1_305_cnt] -> Mux2/60
  [IO_CAN1_301_cnt] -> Mux2/57
  [IO_CAN1_302_cnt] -> Mux2/58
  [IO_CAN1_303_cnt] -> Mux2/59
  [IN_CAN2_542_Fault] -> Mux2/43
  [IN_CAN2_541_Fault] -> Mux2/42
  [IN_CAN2_540_Fault] -> Mux2/41
  [IN_CAN2_543_Fault] -> Mux2/44
  [IO_CAN1_305_cnt] -> Mux2/48
  [IO_CAN1_301_cnt] -> Mux2/45
  [IO_CAN1_302_cnt] -> Mux2/46
  [IO_CAN1_303_cnt] -> Mux2/47
  [IO_CAN2_538_Age] -> Mux2/39
  [IO_CAN2_537_Age] -> Mux2/38
  [IO_CAN2_536_Age] -> Mux2/37
  [IN_CAN2_539_Fault] -> Mux2/40
  [IO_CAN2_535_Age] -> Mux2/36
  [IO_CAN2_532_Age] -> Mux2/33
  [IO_CAN2_533_Age] -> Mux2/34
  [IO_CAN2_534_Age] -> Mux2/35
  Demux1/2 -> [IN_CAN2_501_Fault], raptor_fault_def1/1
  Demux1/4 -> raptor_fault_def3/1, [IN_CAN2_503_Fault]
  Demux1/3 -> [IN_CAN2_502_Fault], raptor_fault_def2/1
  Demux1/7 -> raptor_fault_def6/1, [IN_CAN2_506_Fault]
  Demux1/8 -> [IN_CAN2_507_Fault], raptor_fault_def7/1
  Demux1/6 -> raptor_fault_def5/1, [IN_CAN2_505_Fault]
  Demux1/5 -> [IN_CAN2_504_Fault], raptor_fault_def4/1
  Demux1/13 -> raptor_fault_def12/1, [IN_CAN2_512_Fault]
  Demux1/14 -> [IN_CAN2_513_Fault], raptor_fault_def13/1
  Demux1/16 -> raptor_fault_def15/1, [IN_CAN2_515_Fault]
  Demux1/15 -> [IN_CAN2_514_Fault], raptor_fault_def14/1
  Demux1/11 -> raptor_fault_def10/1, [IN_CAN2_510_Fault]
  Demux1/12 -> [IN_CAN2_511_Fault], raptor_fault_def11/1
  Demux1/10 -> raptor_fault_def9/1, [IN_CAN2_509_Fault]
  Demux1/9 -> [IN_CAN2_508_Fault], raptor_fault_def8/1
  Demux1/25 -> raptor_fault_def30/1, [IN_CAN2_524_Fault]
  Demux1/26 -> [IN_CAN2_525_Fault], raptor_fault_def31/1
  Demux1/28 -> raptor_fault_def19/1, [IN_CAN2_527_Fault]
  Demux1/27 -> [IN_CAN2_526_Fault], raptor_fault_def18/1
  Demux1/31 -> raptor_fault_def22/1, [IN_CAN2_530_Fault]
  Demux1/30 -> raptor_fault_def21/1, [IN_CAN2_529_Fault]
  Demux1/29 -> [IN_CAN2_528_Fault], raptor_fault_def20/1
  Demux1/21 -> raptor_fault_def26/1, [IN_CAN2_520_Fault]
  Demux1/22 -> [IN_CAN2_521_Fault], raptor_fault_def27/1
  Demux1/24 -> raptor_fault_def29/1, [IN_CAN2_523_Fault]
  Demux1/23 -> [IN_CAN2_522_Fault], raptor_fault_def28/1
  Demux1/19 -> raptor_fault_def24/1, [IN_CAN2_518_Fault]
  Demux1/20 -> [IN_CAN2_519_Fault], raptor_fault_def25/1
  Demux1/18 -> raptor_fault_def17/1, [IN_CAN2_517_Fault]
  Demux1/17 -> [IN_CAN2_516_Fault], raptor_fault_def16/1
  Demux1/48 -> raptor_fault_def40/1, [IN_CAN2_547_Fault]
  Demux1/49 -> [IN_CAN2_548_Fault], raptor_fault_def41/1
  Demux1/51 -> raptor_fault_def50/1, [IN_CAN2_550_Fault]
  Demux1/50 -> [IN_CAN2_549_Fault], raptor_fault_def49/1
  Demux1/54 -> raptor_fault_def53/1, [IN_CAN2_553_Fault]
  Demux1/55 -> [IN_CAN2_554_Fault], raptor_fault_def54/1
  Demux1/53 -> raptor_fault_def52/1, [IN_CAN2_552_Fault]
  Demux1/52 -> [IN_CAN2_551_Fault], raptor_fault_def51/1
  Demux1/60 -> raptor_fault_def45/1, [IN_CAN2_559_Fault]
  Demux1/61 -> [IN_CAN2_560_Fault], raptor_fault_def46/1
  Demux1/63 -> raptor_fault_def48/1, [IN_CAN2_562_Fault]
  Demux1/62 -> [IN_CAN2_561_Fault], raptor_fault_def47/1
  Demux1/58 -> raptor_fault_def42/1, [IN_CAN2_557_Fault]
  Demux1/59 -> [IN_CAN2_558_Fault], raptor_fault_def43/1
  Demux1/57 -> raptor_fault_def57/1, [IN_CAN2_556_Fault]
  Demux1/56 -> [IN_CAN2_555_Fault], raptor_fault_def56/1
  Demux1/40 -> raptor_fault_def62/1, [IN_CAN2_539_Fault]
  Demux1/41 -> [IN_CAN2_540_Fault], raptor_fault_def63/1
  Demux1/43 -> raptor_fault_def35/1, [IN_CAN2_542_Fault]
  Demux1/42 -> [IN_CAN2_541_Fault], raptor_fault_def34/1
  Demux1/46 -> raptor_fault_def38/1, [IN_CAN2_545_Fault]
  Demux1/47 -> [IN_CAN2_546_Fault], raptor_fault_def39/1
  Demux1/45 -> raptor_fault_def37/1, [IN_CAN2_544_Fault]
  Demux1/44 -> [IN_CAN2_543_Fault], raptor_fault_def36/1
  Demux1/36 -> raptor_fault_def58/1, [IN_CAN2_535_Fault]
  Demux1/37 -> [IN_CAN2_536_Fault], raptor_fault_def59/1
  Demux1/39 -> raptor_fault_def61/1, [IN_CAN2_538_Fault]
  Demux1/38 -> [IN_CAN2_537_Fault], raptor_fault_def60/1
  Demux1/34 -> raptor_fault_def44/1, [IN_CAN2_533_Fault]
  Demux1/35 -> [IN_CAN2_534_Fault], raptor_fault_def55/1
  Demux1/33 -> raptor_fault_def33/1, [IN_CAN2_532_Fault]
  Demux1/32 -> raptor_fault_def23/1, [IN_CAN2_531_Fault]
  IO_CAN2_500_Bus/1 -> Bus Selector/1  "IO_CAN2_500_Bus"
  Bus Selector/1 -> [IO_CAN2_500_Age]  "<Age>"
  Bus Selector/5 -> [IO_CAN2_500_cnt]  "<BMS_rollingMsg500>"
  OverMeas/1 -> ?  "IN_PackCurrent_A"
  Demux2/2 -> OverMeas1/1
  Switch/1 -> Demux2/1
  [IN_CAN2_500_Fault] -> Switch/2
  Mux3/1 -> Switch/3
  OverMeas1/1 -> ?  "IN_PackSOC_pct"
  Demux2/1 -> OverMeas/1
  Constant/1 -> Switch/1
  Bus Selector/2 -> Mux3/1  "<BMS_packCurr>"
  Bus Selector/3 -> Mux3/2  "<BMS_packSOC>"
  Bus Selector/4 -> Mux3/3  "<BMS_packVoltage>"
  OverMeas2/1 -> ?  "IN_PackVoltage_V"
  Demux2/3 -> OverMeas2/1
  Demux3/3 -> OverMeas5/1
  OverMeas5/1 -> ?  "IN_module3V_V"
  Constant1/1 -> Switch1/1
  Demux3/1 -> OverMeas3/1
  OverMeas4/1 -> ?  "IN_module2V_V"
  Mux4/1 -> Switch1/3
  [IN_CAN2_501_Fault] -> Switch1/2
  Switch1/1 -> Demux3/1
  Demux3/2 -> OverMeas4/1
  OverMeas3/1 -> ?  "IN_module1V_V"
  IO_CAN2_501_Bus/1 -> Bus Selector1/1  "IO_CAN2_500_Bus"
  Bus Selector1/1 -> [IO_CAN2_501_Age]  "<Age>"
  Bus Selector1/5 -> [IO_CAN2_501_cnt]  "<BMS_counterMsg501>"
  Bus Selector1/2 -> Mux4/1  "<BMS_module1V>"
  Bus Selector1/3 -> Mux4/2  "<BMS_module2V>"
  Bus Selector1/4 -> Mux4/3  "<BMS_module3V>"
  IO_CAN2_502_Bus/1 -> Bus Selector2/1  "IO_CAN2_502_Bus"
  OverMeas6/1 -> ?  "IN_module4V_V"
  Demux4/2 -> OverMeas7/1
  Switch2/1 -> Demux4/1
  [IN_CAN2_502_Fault] -> Switch2/2
  Mux5/1 -> Switch2/3
  OverMeas7/1 -> ?  "IN_module5V_V"
  Demux4/1 -> OverMeas6/1
  Constant2/1 -> Switch2/1
  Demux7/3 -> OverMeas17/1
  OverMeas17/1 -> ?  "IN_module1Cell9Volt_V"
  Constant5/1 -> Switch5/1
  Demux7/1 -> OverMeas15/1
  OverMeas16/1 -> ?  "IN_module1Cell8Volt_V"
  Mux8/1 -> Switch5/3
  [IN_CAN2_505_Fault] -> Switch5/2
  Switch5/1 -> Demux7/1
  Demux7/2 -> OverMeas16/1
  OverMeas15/1 -> ?  "IN_module1Cell7Volt_V"
  IO_CAN2_505_Bus/1 -> Bus Selector5/1  "IO_CAN2_505_Bus"
  IO_CAN2_504_Bus/1 -> Bus Selector4/1  "IO_CAN2_504_Bus"
  OverMeas12/1 -> ?  "IN_module1Cell4Volt_V"
  Demux6/2 -> OverMeas13/1
  Switch4/1 -> Demux6/1
  [IN_CAN2_504_Fault] -> Switch4/2
  Mux7/1 -> Switch4/3
  OverMeas13/1 -> ?  "IN_module1Cell5Volt_V"
  Demux6/1 -> OverMeas12/1
  Constant4/1 -> Switch4/1
  OverMeas14/1 -> ?  "IN_module1Cell6Volt_V"
  Demux6/3 -> OverMeas14/1
  Demux5/3 -> OverMeas11/1
  OverMeas11/1 -> ?  "IN_module1Cell3Volt_V"
  Constant3/1 -> Switch3/1
  Demux5/1 -> OverMeas9/1
  OverMeas10/1 -> ?  "IN_module1Cell2Volt_V"
  Mux6/1 -> Switch3/3
  [IN_CAN2_503_Fault] -> Switch3/2
  Switch3/1 -> Demux5/1
  Demux5/2 -> OverMeas10/1
  OverMeas9/1 -> ?  "IN_module1Cell1Volt_V"
  Bus Selector3/1 -> [IO_CAN2_503_Age]  "<Age>"
  IO_CAN2_503_Bus/1 -> Bus Selector3/1  "IO_CAN2_503_Bus"
  Bus Selector3/5 -> [IO_CAN2_503_cnt]  "<BMS_counterMsg503>"
  Bus Selector3/4 -> Mux6/3  "<BMS_module1Cell3Volt>"
  Bus Selector4/1 -> [IO_CAN2_504_Age]  "<Age>"
  Bus Selector4/5 -> [IO_CAN2_504_cnt]  "<BMS_counterMsg504>"
  Bus Selector5/5 -> [IO_CAN2_505_cnt]  "<BMS_counterMsg505>"
  Bus Selector2/1 -> [IO_CAN2_502_Age]  "<Age>"
  Bus Selector2/2 -> Mux5/1  "<BMS_module4V>"
  Bus Selector2/3 -> Mux5/2  "<BMS_module5V>"
  Bus Selector2/4 -> [IO_CAN2_502_cnt]  "<BMS_counterMsg502>"
  IO_CAN2_507_Bus/1 -> Bus Selector7/1  "IO_CAN2_507_Bus"
  OverMeas27/1 -> ?  "IN_module1Cell13Volt_V"
  Demux9/2 -> OverMeas8/1
  Switch7/1 -> Demux9/1
  [IN_CAN2_507_Fault] -> Switch7/2
  Mux10/1 -> Switch7/3
  OverMeas8/1 -> ?  "IN_module1Cell14Volt_V"
  Demux9/1 -> OverMeas27/1
  Constant7/1 -> Switch7/1
  OverMeas18/1 -> ?  "IN_module1Cell15Volt_V"
  Demux9/3 -> OverMeas18/1
  Constant8/1 -> Switch8/1
  OverMeas20/1 -> ?  "IN_module1Cell18V_V"
  Mux11/1 -> Switch8/3
  [IN_CAN2_508_Fault] -> Switch8/2
  Switch8/1 -> Demux10/1
  OverMeas19/1 -> ?  "IN_module1Cell17V_V"
  IO_CAN2_508_Bus/1 -> Bus Selector8/1  "IO_CAN2_508_Bus"
  IO_CAN2_509_Bus/1 -> Bus Selector9/1  "IO_CAN2_509_Bus"
  OverMeas22/1 -> ?  "IN_module1Cell1Temp_degC"
  Demux11/2 -> OverMeas23/1
  Switch9/1 -> Demux11/1
  [IN_CAN2_509_Fault] -> Switch9/2
  Mux12/1 -> Switch9/3
  OverMeas23/1 -> ?  "IN_module1Cell2Temp_degC"
  Demux11/1 -> OverMeas22/1
  Constant9/1 -> Switch9/1
  OverMeas24/1 -> ?  "IN_module1Cell3Temp_degC"
  Demux11/3 -> OverMeas24/1
  Constant6/1 -> Switch6/1
  Demux12/1 -> OverMeas25/1
  OverMeas26/1 -> ?  "IN_module1Cell11Volt_V"
  Mux9/1 -> Switch6/3
  [IN_CAN2_506_Fault] -> Switch6/2
  Switch6/1 -> Demux12/1
  Demux12/2 -> OverMeas26/1
  OverMeas25/1 -> ?  "IN_module1Cell10Volt_V"
  IO_CAN2_506_Bus/1 -> Bus Selector6/1  "IO_CAN2_506_Bus"
  Bus Selector6/1 -> [IO_CAN2_506_Age]  "<Age>"
  Bus Selector6/5 -> [IO_CAN2_506_cnt]  "<BMS_counterMsg506>"
  Demux12/3 -> OverMeas28/1
  OverMeas28/1 -> ?  "IN_module1Cell12Volt_V"
  Bus Selector7/1 -> [IO_CAN2_507_Age]  "<Age>"
  Bus Selector7/5 -> [IO_CAN2_507_cnt]  "<BMS_counterMsg507>"
  Bus Selector8/1 -> [IO_CAN2_508_Age]  "<Age>"
  Bus Selector8/5 -> [IO_CAN2_508_cnt]  "<BMS_counterMsg508>"
  Bus Selector9/1 -> [IO_CAN2_509_Age]  "<Age>"
  OverMeas34/1 -> ?  "IN_module1Cell9Temp_degC"
  OverMeas31/1 -> ?  "IN_module1Cell6Temp_degC"
  OverMeas33/1 -> ?  "IN_module1Cell8Temp_degC"
  OverMeas30/1 -> ?  "IN_module1Cell5Temp_degC"
  OverMeas37/1 -> ?  "IN_module1Cell11Temp_degC"
  OverMeas36/1 -> ?  "IN_module1Cell10Temp_degC"
  Demux14/3 -> OverMeas34/1
  Mux14/1 -> Switch10/3
  OverMeas39/1 -> ?  "IN_module1Cell12Temp_degC"
  IO_CAN2_511_Bus/1 -> Bus Selector11/1  "IO_CAN2_511_Bus"
  OverMeas32/1 -> ?  "IN_module1Cell7Temp_degC"
  Constant10/1 -> Switch10/1
  Switch11/1 -> Demux14/1
  Demux8/3 -> OverMeas39/1
  IO_CAN2_510_Bus/1 -> Bus Selector39/1  "IO_CAN2_510_Bus"
  Demux13/1 -> OverMeas29/1
  Constant12/1 -> Switch12/1
  Mux15/1 -> Switch11/3
  Constant11/1 -> Switch11/1
  Demux14/2 -> OverMeas33/1
  Mux16/1 -> Switch12/3
  Switch10/1 -> Demux13/1
  [IN_CAN2_510_Fault] -> Switch10/2
  Demux14/1 -> OverMeas32/1
  Demux8/1 -> OverMeas36/1
  Demux13/2 -> OverMeas30/1
  Demux13/3 -> OverMeas31/1
  IO_CAN2_512_Bus/1 -> Bus Selector12/1  "IO_CAN2_512_Bus"
  [IN_CAN2_512_Fault] -> Switch12/2
  Demux8/2 -> OverMeas37/1
  OverMeas29/1 -> ?  "IN_module1Cell4Temp_degC"
  [IN_CAN2_511_Fault] -> Switch11/2
  Switch12/1 -> Demux8/1
  OverMeas38/1 -> ?  "IN_module1Cell14Temp_degC"
  OverMeas40/1 -> ?  "IN_module1Cell15Temp_degC"
  OverMeas35/1 -> ?  "IN_module1Cell13Temp_degC"
  Mux13/1 -> Switch13/3
  Constant13/1 -> Switch13/1
  Demux15/3 -> OverMeas40/1
  Switch13/1 -> Demux15/1
  Demux15/1 -> OverMeas35/1
  [IN_CAN2_513_Fault] -> Switch13/2
  IO_CAN2_513_Bus/1 -> Bus Selector14/1  "IO_CAN2_513_Bus"
  Demux15/2 -> OverMeas38/1
  Bus Selector12/1 -> [IO_CAN2_512_Age]  "<Age>"
  Bus Selector12/5 -> [IO_CAN2_512_cnt]  "<BMS_counterMsg512>"
  Bus Selector14/1 -> [IO_CAN2_513_Age]  "<Age>"
  Bus Selector14/2 -> Mux13/1  "<BMS_module1Cell10Temp>"
  Bus Selector14/3 -> Mux13/2  "<BMS_module1Cell11Temp>"
  Bus Selector14/4 -> Mux13/3  "<BMS_module1Cell12Temp>"
  Bus Selector14/5 -> [IO_CAN2_513_cnt]  "<BMS_counterMsg512>"
  OverMeas41/1 -> ?  "IN_module1Cell17Temp_degC"
  OverMeas21/1 -> ?  "IN_module1Cell16Temp_degC"
  Mux17/1 -> Switch14/3
  Constant14/1 -> Switch14/1
  Switch14/1 -> Demux16/1
  Demux16/1 -> OverMeas21/1
  [IN_CAN2_514_Fault] -> Switch14/2
  IO_CAN2_514_Bus/1 -> Bus Selector13/1  "IO_CAN2_514_Bus"
  Demux16/2 -> OverMeas41/1
  Bus Selector13/5 -> [IO_CAN2_514_cnt]  "<BMS_counterMsg514>"
  OverMeas49/1 -> ?  "IN_module2Cell9V_V"
  OverMeas43/1 -> ?  "IN_module2Cell3V_V"
  OverMeas47/1 -> ?  "IN_module2Cell7V_V"
  OverMeas44/1 -> ?  "IN_module2Cell4V_V"
  OverMeas45/1 -> ?  "IN_module2Cell5V_V"
  OverMeas42/1 -> ?  "IN_module2Cell2V_V"
  OverMeas55/1 -> ?  "IN_module2Cell13V_V"
  OverMeas58/1 -> ?  "IN_module2Cell1V_V"
  OverMeas57/1 -> ?  "IN_module2Cell14V_V"
  OverMeas52/1 -> ?  "IN_module2Cell18V_V"
  OverMeas51/1 -> ?  "IN_module2Cell17V_V"
  OverMeas50/1 -> ?  "IN_module2Cell15V_V"
  OverMeas54/1 -> ?  "IN_module2Cell11V_V"
  OverMeas53/1 -> ?  "IN_module2Cell10V_V"
  Constant15/1 -> Switch15/1
  IO_CAN2_515_Bus/1 -> Bus Selector15/1  "IO_CAN2_515_Bus"
  Demux19/3 -> OverMeas43/1
  Mux19/1 -> Switch20/3
  OverMeas46/1 -> ?  "IN_module2Cell6V_V"
  Demux21/3 -> OverMeas49/1
  Mux21/1 -> Switch16/3
  OverMeas56/1 -> ?  "IN_module2Cell12V_V"
  Constant20/1 -> Switch20/1
  Constant19/1 -> Switch19/1
  Demux19/2 -> OverMeas42/1
  Switch20/1 -> Demux17/1
  OverMeas48/1 -> ?  "IN_module2Cell8V_V"
  IO_CAN2_517_Bus/1 -> Bus Selector17/1  "IO_CAN2_517_Bus"
  Bus Selector17/2 -> Mux22/1  "<BMS_module1seg7V>"
  Bus Selector17/1 -> [IO_CAN2_517_Age]  "<Age>"
  Mux18/1 -> Switch19/3
  Constant16/1 -> Switch16/1
  IO_CAN2_516_Bus/1 -> Bus Selector16/1  "IO_CAN2_516_Bus"
  Demux18/3 -> OverMeas56/1
  Switch17/1 -> Demux21/1
  Bus Selector17/4 -> Mux22/3  "<BMS_module1seg9V>"
  Demux20/1 -> OverMeas44/1
  Constant18/1 -> Switch18/1
  Demux19/1 -> OverMeas58/1
  Bus Selector17/5 -> [IO_CAN2_517_cnt]  "<BMS_counterMsg504>"
  Demux22/3 -> OverMeas50/1
  Constant17/1 -> Switch17/1
  IO_CAN2_519_Bus/1 -> Bus Selector19/1  "IO_CAN2_519_Bus"
  Bus Selector17/3 -> Mux22/2  "<BMS_module1seg8V>"
  Demux21/2 -> OverMeas48/1
  [IN_CAN2_515_Fault] -> Switch15/2
  Mux23/1 -> Switch18/3
  IO_CAN2_520_Bus/1 -> Bus Selector20/1  "IO_CAN2_520_Bus"
  [IN_CAN2_520_Fault] -> Switch20/2
  Switch16/1 -> Demux20/1
  Switch15/1 -> Demux19/1
  Mux20/1 -> Switch15/3
  [IN_CAN2_516_Fault] -> Switch16/2
  Demux21/1 -> OverMeas47/1
  Demux18/1 -> OverMeas53/1
  Demux20/2 -> OverMeas45/1
  Demux22/2 -> OverMeas57/1
  IO_CAN2_518_Bus/1 -> Bus Selector18/1  "IO_CAN2_518_Bus"
  [IN_CAN2_518_Fault] -> Switch18/2
  Demux20/3 -> OverMeas46/1
  Switch19/1 -> Demux22/1
  Demux22/1 -> OverMeas55/1
  Mux22/1 -> Switch17/3
  Demux18/2 -> OverMeas54/1
  Switch18/1 -> Demux18/1
  [IN_CAN2_519_Fault] -> Switch19/2
  [IN_CAN2_517_Fault] -> Switch17/2
  Bus Selector16/1 -> [IO_CAN2_516_Age]  "<Age>"
  Bus Selector16/2 -> Mux21/1  "<BMS_module2seg4V>"
  Bus Selector16/3 -> Mux21/2  "<BMS_module2seg5V>"
  Bus Selector16/4 -> Mux21/3  "<BMS_module2seg6V>"
  Bus Selector16/5 -> [IO_CAN2_516_cnt]  "<BMS_counterMsg516>"
  Bus Selector18/1 -> [IO_CAN2_518_Age]  "<Age>"
  Bus Selector18/5 -> [IO_CAN2_518_cnt]  "<BMS_counterMsg518>"
  Bus Selector18/4 -> Mux23/3  "<BMS_module2seg12V>"
  Bus Selector18/3 -> Mux23/2  "<BMS_module2seg11V>"
  Bus Selector18/2 -> Mux23/1  "<BMS_module2seg10V>"
  Bus Selector19/1 -> [IO_CAN2_519_Age]  "<Age>"
  Bus Selector19/2 -> Mux18/1  "<BMS_module2seg13V>"
  Bus Selector19/3 -> Mux18/2  "<BMS_module2seg14V>"
  Bus Selector19/4 -> Mux18/3  "<BMS_module2seg15V>"
  Bus Selector19/5 -> [IO_CAN2_519_cnt]  "<BMS_counterMsg519>"
  Bus Selector20/1 -> [IO_CAN2_520_Age]  "<Age>"
  Bus Selector20/2 -> Mux19/1  "<BMS_module2seg16V>"
  Bus Selector20/5 -> [IO_CAN2_520_cnt]  "<BMS_counterMsg520>"
  Bus Selector20/3 -> Mux19/2  "<BMS_module2seg17V>"
  Bus Selector20/4 -> Mux19/3  "<BMS_module2seg18V>"
  OverMeas59/1 -> ?  "IN_module1Cell18Temp_degC"
  Demux16/3 -> OverMeas59/1
  Bus Selector15/1 -> [IO_CAN2_515_Age]  "<Age>"
  Bus Selector15/2 -> Mux20/1  "<BMS_module2seg1V>"
  Bus Selector15/3 -> Mux20/2  "<BMS_module2seg2V>"
  Bus Selector15/4 -> Mux20/3  "<BMS_module2seg3V>"
  Bus Selector15/5 -> [IO_CAN2_515_cnt]  "<BMS_counterMsg515>"
  OverMeas80/1 -> ?  "IN_module2Cell18Temp_degC"
  IO_CAN2_525_Bus/1 -> Bus Selector25/1  "IO_CAN2_525_Bus"
  IO_CAN2_524_Bus/1 -> Bus Selector23/1  "IO_CAN2_524_Bus"
  Demux26/2 -> OverMeas73/1
  Switch24/1 -> Demux26/1
  Constant24/1 -> Switch24/1
  Demux26/1 -> OverMeas70/1
  OverMeas75/1 -> ?  "IN_module2Cell15Temp_degC"
  OverMeas70/1 -> ?  "IN_module2Cell13Temp_degC"
  IO_CAN2_523_Bus/1 -> Bus Selector22/1  "IO_CAN2_523_Bus"
  [IN_CAN2_523_Fault] -> Switch22/2
  Switch23/1 -> Demux29/1
  Demux29/2 -> OverMeas72/1
  [IN_CAN2_524_Fault] -> Switch23/2
  Demux25/2 -> OverMeas68/1
  Mux28/1 -> Switch23/3
  Demux24/2 -> OverMeas65/1
  Switch21/1 -> Demux24/1
  Demux25/1 -> OverMeas67/1
  Demux29/1 -> OverMeas71/1
  [IN_CAN2_522_Fault] -> Switch21/2
  Constant22/1 -> Switch22/1
  IO_CAN2_522_Bus/1 -> Bus Selector21/1  "IO_CAN2_522_Bus"
  Demux24/1 -> OverMeas64/1
  Mux27/1 -> Switch22/3
  Constant23/1 -> Switch23/1
  Switch22/1 -> Demux25/1
  Demux29/3 -> OverMeas74/1
  Constant21/1 -> Switch21/1
  Demux26/3 -> OverMeas75/1
  OverMeas67/1 -> ?  "IN_module2Cell7Temp_degC"
  Mux26/1 -> Switch21/3
  Demux25/3 -> OverMeas69/1
  OverMeas72/1 -> ?  "IN_module2Cell11Temp_degC"
  OverMeas69/1 -> ?  "IN_module2Cell9Temp_degC"
  OverMeas65/1 -> ?  "IN_module2Cell5Temp_degC"
  Bus Selector26/1 -> [IO_CAN2_527_Age]  "<Age>"
  OverMeas74/1 -> ?  "IN_module2Cell12Temp_degC"
  OverMeas68/1 -> ?  "IN_module2Cell8Temp_degC"
  Demux27/2 -> OverMeas76/1
  OverMeas71/1 -> ?  "IN_module2Cell10Temp_degC"
  IO_CAN2_526_Bus/1 -> Bus Selector24/1  "IO_CAN2_526_Bus"
  Constant25/1 -> Switch25/1
  Demux27/1 -> OverMeas60/1
  Switch25/1 -> Demux27/1
  Demux27/3 -> OverMeas80/1
  OverMeas62/1 -> ?  "IN_module2Cell2Temp_degC"
  OverMeas63/1 -> ?  "IN_module2Cell3Temp_degC"
  Bus Selector21/1 -> [IO_CAN2_522_Age]  "<Age>"
  IO_CAN2_521_Bus/1 -> Bus Selector27/1  "IO_CAN2_521_Bus"
  Mux29/1 -> Switch25/3
  Switch27/1 -> Demux23/1
  OverMeas60/1 -> ?  "IN_module2Cell16Temp_degC"
  Demux24/3 -> OverMeas66/1
  Demux23/3 -> OverMeas63/1
  [IN_CAN2_521_Fault] -> Switch27/2
  [IN_CAN2_526_Fault] -> Switch25/2
  Constant26/1 -> Switch26/1
  Constant27/1 -> Switch27/1
  OverMeas66/1 -> ?  "IN_module2Cell6Temp_degC"
  Demux23/2 -> OverMeas62/1
  IO_CAN2_527_Bus/1 -> Bus Selector26/1  "IO_CAN2_527_Bus"
  Demux23/1 -> OverMeas61/1
  Mux24/1 -> Switch27/3
  OverMeas64/1 -> ?  "IN_module2Cell4Temp_degC"
  Demux28/3 -> OverMeas78/1
  OverMeas77/1 -> ?  "IN_module3Cell2V_V"
  OverMeas78/1 -> ?  "IN_module3Cell3V_V"
  Mux30/1 -> Switch26/3
  OverMeas76/1 -> ?  "IN_module2Cell17Temp_degC"
  Switch26/1 -> Demux28/1
  OverMeas73/1 -> ?  "IN_module2Cell14Temp_degC"
  [IN_CAN2_527_Fault] -> Switch26/2
  Demux28/1 -> OverMeas79/1
  Demux28/2 -> OverMeas77/1
  OverMeas79/1 -> ?  "IN_module3Cell1V_V"
  [IN_CAN2_525_Fault] -> Switch24/2
  OverMeas61/1 -> ?  "IN_module2Cell1Temp_degC"
  Mux25/1 -> Switch24/3
  Demux17/2 -> OverMeas51/1
  Demux17/3 -> OverMeas52/1
  OverMeas81/1 -> ?  "IN_module2Cell16V_V"
  Demux17/1 -> OverMeas81/1
  Bus Selector25/1 -> [IO_CAN2_525_Age]  "<Age>"
  IO_CAN2_530_Bus/1 -> Bus Selector30/1  "IO_CAN2_530_Bus"
  OverMeas85/1 -> ?  "IN_module3Cell7V_V"
  OverMeas93/1 -> ?  "IN_module3Cell13V_V"
  IO_CAN2_528_Bus/1 -> Bus Selector28/1  "IO_CAN2_528_Bus"
  OverMeas91/1 -> ?  "IN_module3Cell10V_V"
  OverMeas92/1 -> ?  "IN_module3Cell11V_V"
  Demux30/2 -> OverMeas89/1
  OverMeas89/1 -> ?  "IN_module3Cell17V_V"
  IO_CAN2_532_Bus/1 -> Bus Selector32/1  "IO_CAN2_532_Bus"
  OverMeas83/1 -> ?  "IN_module3Seg5V_V"
  IO_CAN2_529_Bus/1 -> Bus Selector29/1  "IO_CAN2_529_Bus"
  Demux32/2 -> OverMeas83/1
  Demux34/2 -> OverMeas95/1
  [IN_CAN2_528_Fault] -> Switch28/2
  Switch28/1 -> Demux32/1
  [IN_CAN2_532_Fault] -> Switch32/2
  OverMeas88/1 -> ?  "IN_module3Cell15V_V"
  Demux33/2 -> OverMeas86/1
  OverMeas95/1 -> ?  "IN_module3Cell14V_V"
  IO_CAN2_531_Bus/1 -> Bus Selector31/1  "IO_CAN2_531_Bus"
  Constant29/1 -> Switch29/1
  Demux32/1 -> OverMeas82/1
  Constant30/1 -> Switch30/1
  Demux31/3 -> OverMeas94/1
  Switch29/1 -> Demux33/1
  Mux31/1 -> Switch31/3
  Demux34/3 -> OverMeas88/1
  Switch32/1 -> Demux30/1
  Constant28/1 -> Switch28/1
  OverMeas86/1 -> ?  "IN_module3Cell8V_V"
  OverMeas94/1 -> ?  "IN_module3Cell12V_V"
  Mux35/1 -> Switch30/3
  Demux33/3 -> OverMeas87/1
  Constant31/1 -> Switch31/1
  Mux33/1 -> Switch28/3
  OverMeas82/1 -> ?  "IN_module3Cell4V_V"
  [IN_CAN2_531_Fault] -> Switch31/2
  [IN_CAN2_529_Fault] -> Switch29/2
  OverMeas84/1 -> ?  "IN_module3Seg6V_V"
  Demux30/1 -> OverMeas96/1
  Demux31/2 -> OverMeas92/1
  Switch30/1 -> Demux31/1
  Demux32/3 -> OverMeas84/1
  Demux31/1 -> OverMeas91/1
  Demux30/3 -> OverMeas90/1
  OverMeas87/1 -> ?  "IN_module3Cell9V_V"
  Mux34/1 -> Switch29/3
  Switch31/1 -> Demux34/1
  Demux34/1 -> OverMeas93/1
  OverMeas96/1 -> ?  "IN_module3Cell16V_V"
  Mux32/1 -> Switch32/3
  Demux33/1 -> OverMeas85/1
  OverMeas90/1 -> ?  "IN_module3Cell18V_V"
  [IN_CAN2_530_Fault] -> Switch30/2
  Constant32/1 -> Switch32/1
  Bus Selector26/2 -> Mux30/1  "<BMS_module3seg1V>"
  Bus Selector26/3 -> Mux30/2  "<BMS_module3seg2V>"
  Bus Selector26/4 -> Mux30/3  "<BMS_module3seg3V>"
  Bus Selector26/5 -> [IO_CAN2_527_cnt]  "<BMS_counterMsg527>"
  Bus Selector30/1 -> [IO_CAN2_530_Age]  "<Age>"
  Bus Selector31/2 -> Mux31/1  "<BMS_module3seg13V>"
  Bus Selector31/3 -> Mux31/2  "<BMS_module3seg14V>"
  Bus Selector31/4 -> Mux31/3  "<BMS_module3seg15V>"
  Bus Selector31/5 -> [IO_CAN2_531_cnt]  "<BMS_counterMsg531>"
  Bus Selector31/1 -> [IO_CAN2_531_Age]  "<Age>"
  Bus Selector32/1 -> [IO_CAN2_532_Age]  "<Age>"
  Bus Selector32/5 -> [IO_CAN2_532_cnt]  "<BMS_counterMsg532>"
  Bus Selector32/2 -> Mux32/1  "<BMS_module3seg16V>"
  Bus Selector32/3 -> Mux32/2  "<BMS_module3seg17V>"
  Bus Selector32/4 -> Mux32/3  "<BMS_module3seg18V>"
  OverMeas97/1 -> ?  "IN_module1Cell16V_V"
  Demux10/1 -> OverMeas97/1
  Demux10/2 -> OverMeas19/1
  Demux10/3 -> OverMeas20/1
  IO_CAN2_536_Bus/1 -> Bus Selector35/1  "IO_CAN2_536_Bus"
  IO_CAN2_533_Bus/1 -> Bus Selector38/1  "IO_CAN2_533_Bus"
  IO_CAN2_535_Bus/1 -> Bus Selector34/1  "IO_CAN2_535_Bus"
  IO_CAN2_538_Bus/1 -> Bus Selector36/1  "IO_CAN2_538_Bus"
  Bus Selector37/1 -> [IO_CAN2_537_Age]  "<Age>"
  OverMeas115/1 -> ?  "IN_module3Cell18Temp_degC"
  OverMeas111/1 -> ?  "IN_module3Cell14Temp_degC"
  Demux35/1 -> OverMeas99/1
  Demux35/2 -> OverMeas100/1
  OverMeas102/1 -> ?  "IN_module3Cell4Temp_degC"
  [IN_CAN2_533_Fault] -> Switch38/2
  Constant38/1 -> Switch38/1
  Switch38/1 -> Demux35/1
  OverMeas114/1 -> ?  "IN_module3Cell17Temp_degC"
  Mux41/1 -> Switch37/3
  Constant37/1 -> Switch37/1
  Mux37/1 -> Switch36/3
  Demux39/1 -> OverMeas98/1
  Demux39/2 -> OverMeas114/1
  OverMeas106/1 -> ?  "IN_module3Cell8Temp_degC"
  OverMeas98/1 -> ?  "IN_module3Cell16Temp_degC"
  OverMeas109/1 -> ?  "IN_module3Cell10Temp_degC"
  OverMeas112/1 -> ?  "IN_module3Cell12Temp_degC"
  OverMeas110/1 -> ?  "IN_module3Cell11Temp_degC"
  Mux38/1 -> Switch33/3
  OverMeas104/1 -> ?  "IN_module3Cell6Temp_degC"
  Demux37/3 -> OverMeas107/1
  Mux36/1 -> Switch38/3
  Demux38/3 -> OverMeas113/1
  OverMeas103/1 -> ?  "IN_module3Cell5Temp_degC"
  Constant33/1 -> Switch33/1
  OverMeas100/1 -> ?  "IN_module3Cell2Temp_degC"
  Demux40/3 -> OverMeas112/1
  OverMeas107/1 -> ?  "IN_module3Cell9Temp_degC"
  [IN_CAN2_538_Fault] -> Switch37/2
  Demux36/1 -> OverMeas102/1
  OverMeas99/1 -> ?  "IN_module3Cell1Temp_degC"
  Constant34/1 -> Switch34/1
  OverMeas105/1 -> ?  "IN_module3Cell7Temp_degC"
  Demux40/1 -> OverMeas109/1
  [IN_CAN2_537_Fault] -> Switch36/2
  [IN_CAN2_534_Fault] -> Switch33/2
  Demux35/3 -> OverMeas101/1
  Switch34/1 -> Demux37/1
  Constant35/1 -> Switch35/1
  Demux37/1 -> OverMeas105/1
  Mux39/1 -> Switch34/3
  Switch33/1 -> Demux36/1
  Switch37/1 -> Demux39/1
  Demux37/2 -> OverMeas106/1
  IO_CAN2_534_Bus/1 -> Bus Selector33/1  "IO_CAN2_534_Bus"
  [IN_CAN2_536_Fault] -> Switch35/2
  Demux36/2 -> OverMeas103/1
  Demux40/2 -> OverMeas110/1
  Demux36/3 -> OverMeas104/1
  [IN_CAN2_535_Fault] -> Switch34/2
  Demux39/3 -> OverMeas115/1
  Mux40/1 -> Switch35/3
  Constant36/1 -> Switch36/1
  IO_CAN2_537_Bus/1 -> Bus Selector37/1  "IO_CAN2_537_Bus"
  Switch35/1 -> Demux40/1
  Switch36/1 -> Demux38/1
  OverMeas108/1 -> ?  "IN_module3Cell13Temp_degC"
  OverMeas113/1 -> ?  "IN_module3Cell15Temp_degC"
  OverMeas101/1 -> ?  "IN_module3Cell3Temp_degC"
  Demux38/1 -> OverMeas108/1
  Demux38/2 -> OverMeas111/1
  Bus Selector3/2 -> Mux6/1  "<BMS_module1Cell1Volt>"
  Bus Selector3/3 -> Mux6/2  "<BMS_module1Cell2Volt>"
  Bus Selector4/2 -> Mux7/1  "<BMS_module1Cell4Volt>"
  Bus Selector4/3 -> Mux7/2  "<BMS_module1Cell5Volt>"
  Bus Selector4/4 -> Mux7/3  "<BMS_module1Cell6Volt>"
  Bus Selector5/1 -> [IO_CAN2_505_Age]  "<Age>"
  Bus Selector5/2 -> Mux8/1  "<BMS_module1Cell7Volt>"
  Bus Selector5/3 -> Mux8/2  "<BMS_module1Cell8Volt>"
  Bus Selector5/4 -> Mux8/3  "<BMS_module1Cell9Volt>"
  Bus Selector6/2 -> Mux9/1  "<BMS_module1Cell10Volt>"
  Bus Selector6/3 -> Mux9/2  "<BMS_module1Cell11Volt>"
  Bus Selector6/4 -> Mux9/3  "<BMS_module1Cell12Volt>"
  Bus Selector7/2 -> Mux10/1  "<BMS_module1Cell13Volt>"
  Bus Selector7/3 -> Mux10/2  "<BMS_module1Cell14Volt>"
  Bus Selector7/4 -> Mux10/3  "<BMS_module1Cell15Volt>"
  Bus Selector8/2 -> Mux11/1  "<BMS_module1Cell16Volt>"
  Bus Selector8/3 -> Mux11/2  "<BMS_module1Cell17Volt>"
  Bus Selector8/4 -> Mux11/3  "<BMS_module1Cell18Volt>"
  Bus Selector9/2 -> Mux12/1  "<BMS_module1Cell1Temp>"
  Bus Selector9/3 -> Mux12/2  "<BMS_module1Cell2Temp>"
  Bus Selector9/4 -> Mux12/3  "<BMS_module1Cell3Temp>"
  Bus Selector9/5 -> [IO_CAN2_509_cnt]  "<BMS_counterMsg509>"
  Bus Selector11/1 -> [IO_CAN2_511_Age]  "<Age>"
  Bus Selector11/2 -> Mux15/1  "<BMS_module1Cell7Temp>"
  Bus Selector11/3 -> Mux15/2  "<BMS_module1Cell8Temp>"
  Bus Selector11/5 -> [IO_CAN2_511_cnt]  "<BMS_counterMsg511>"
  Bus Selector11/4 -> Mux15/3  "<BMS_module1Cell9Temp>"
  Bus Selector12/2 -> Mux16/1  "<BMS_module1Cell10Temp>"
  Bus Selector12/3 -> Mux16/2  "<BMS_module1Cell11Temp>"
  Bus Selector12/4 -> Mux16/3  "<BMS_module1Cell12Temp>"
  Bus Selector13/1 -> [IO_CAN2_514_Age]  "<Age>"
  Bus Selector13/2 -> Mux17/1  "<BMS_module1Cell16Temp>"
  Bus Selector13/3 -> Mux17/2  "<BMS_module1Cell17Temp>"
  Bus Selector13/4 -> Mux17/3  "<BMS_module1Cell18Temp>"
  Bus Selector39/1 -> [IO_CAN2_510_Age]  "<Age>"
  Bus Selector39/2 -> Mux14/1  "<BMS_module1Cell4Temp>"
  Bus Selector39/3 -> Mux14/2  "<BMS_module1Cell5Temp>"
  Bus Selector39/4 -> Mux14/3  "<BMS_module1Cell6Temp>"
  Bus Selector39/5 -> [IO_CAN2_510_cnt]  "<BMS_counterMsg510>"
  Bus Selector33/1 -> [IO_CAN2_534_Age]  "<Age>"
  Bus Selector33/5 -> [IO_CAN2_534_cnt]  "<BMS_counterMsg534>"
  Bus Selector33/2 -> Mux38/1  "<BMS_module3Cell4Temp>"
  Bus Selector33/3 -> Mux38/2  "<BMS_module3Cell5Temp>"
  Bus Selector33/4 -> Mux38/3  "<BMS_module3Cell6Temp>"
  Bus Selector34/1 -> [IO_CAN2_535_Age]  "<Age>"
  Bus Selector34/5 -> [IO_CAN2_535_cnt]  "<BMS_counterMsg535>"
  Bus Selector34/4 -> Mux39/3  "<BMS_module3Cell9Temp>"
  Bus Selector34/3 -> Mux39/2  "<BMS_module3Cell8Temp>"
  Bus Selector34/2 -> Mux39/1  "<BMS_module3Cell7Temp>"
  Bus Selector35/1 -> [IO_CAN2_536_Age]  "<Age>"
  Bus Selector35/2 -> Mux40/1  "<BMS_module3Cell10Temp>"
  Bus Selector35/3 -> Mux40/2  "<BMS_module3Cell11Temp>"
  Bus Selector35/4 -> Mux40/3  "<BMS_module3Cell12Temp>"
  Bus Selector35/5 -> [IO_CAN2_536_cnt]  "<BMS_counterMsg536>"
  Bus Selector36/1 -> [IO_CAN2_538_Age]  "<Age>"
  Bus Selector36/2 -> Mux41/1  "<BMS_module3Cell16Temp>"
  Bus Selector36/3 -> Mux41/2  "<BMS_module3Cell17Temp>"
  Bus Selector36/4 -> Mux41/3  "<BMS_module3Cell18Temp>"
  Bus Selector36/5 -> [IO_CAN2_538_cnt]  "<BMS_counterMsg538>"
  Bus Selector27/5 -> [IO_CAN2_521_cnt]  "<BMS_counterMsg521>"
  Bus Selector27/1 -> [IO_CAN2_521_Age]  "<Age>"
  Bus Selector27/2 -> Mux24/1  "<BMS_module2Cell1Temp>"
  Bus Selector27/3 -> Mux24/2  "<BMS_module2Cell2Temp>"
  Bus Selector27/4 -> Mux24/3  "<BMS_module2Cell3Temp>"
  Bus Selector37/2 -> Mux37/1  "<BMS_module3Cell13Temp>"
  Bus Selector37/3 -> Mux37/2  "<BMS_module3Cell14Temp>"
  Bus Selector37/4 -> Mux37/3  "<BMS_module3Cell15Temp>"
  Bus Selector37/5 -> [IO_CAN2_537_cnt]  "<BMS_counterMsg537>"
  Bus Selector28/1 -> [IO_CAN2_528_Age]  "<Age>"
  Bus Selector28/2 -> Mux33/1  "<BMS_module3Cell4Volt>"
  Bus Selector28/3 -> Mux33/2  "<BMS_module3Cell5Volt>"
  Bus Selector28/4 -> Mux33/3  "<BMS_module3Cell6Volt>"
  Bus Selector28/5 -> [IO_CAN2_528_cnt]  "<BMS_counterMsg528>"
  Bus Selector29/1 -> [IO_CAN2_529_Age]  "<Age>"
  Bus Selector29/2 -> Mux34/1  "<BMS_module3Cell7Volt>"
  Bus Selector29/3 -> Mux34/2  "<BMS_module3Cell8Volt>"
  Bus Selector29/4 -> Mux34/3  "<BMS_module3Cell9Volt>"
  Bus Selector29/5 -> [IO_CAN2_529_cnt]  "<BMS_counterMsg529>"
  Bus Selector30/2 -> Mux35/1  "<BMS_module3Cell10Volt>"
  Bus Selector30/3 -> Mux35/2  "<BMS_module3Cell11Volt>"
  Bus Selector30/4 -> Mux35/3  "<BMS_module3Cell12Volt>"
  Bus Selector30/5 -> [IO_CAN2_530_cnt]  "<BMS_counterMsg530>"
  Bus Selector21/5 -> [IO_CAN2_522_cnt]  "<BMS_counterMsg522>"
  Bus Selector21/4 -> Mux26/3  "<BMS_module2Cell6Temp>"
  Bus Selector21/3 -> Mux26/2  "<BMS_module2Cell5Temp>"
  Bus Selector21/2 -> Mux26/1  "<BMS_module2Cell4Temp>"
  Bus Selector22/2 -> Mux27/1  "<BMS_module2Cell7Temp>"
  Bus Selector22/3 -> Mux27/2  "<BMS_module2Cell8Temp>"
  Bus Selector22/4 -> Mux27/3  "<BMS_module2Cell9Temp>"
  Bus Selector22/5 -> [IO_CAN2_523_cnt]  "<BMS_counterMsg523>"
  Bus Selector22/1 -> [IO_CAN2_523_Age]  "<Age>"
  Bus Selector23/1 -> [IO_CAN2_524_Age]  "<Age>"
  Bus Selector23/2 -> Mux28/1  "<BMS_module2Cell10Temp>"
  Bus Selector23/3 -> Mux28/2  "<BMS_module2Cell11Temp>"
  Bus Selector23/4 -> Mux28/3  "<BMS_module2Cell12Temp>"
  Bus Selector23/5 -> [IO_CAN2_524_cnt]  "<BMS_counterMsg524>"
  Bus Selector25/2 -> Mux25/1  "<BMS_module2Cell13Temp>"
  Bus Selector25/3 -> Mux25/2  "<BMS_module2Cell14Temp>"
  Bus Selector25/4 -> Mux25/3  "<BMS_module2Cell15Temp>"
  Bus Selector25/5 -> [IO_CAN2_525_cnt]  "<BMS_counterMsg525>"
  Bus Selector24/1 -> [IO_CAN2_526_Age]  "<Age>"
  Bus Selector24/2 -> Mux29/1  "<BMS_module2Cell16Temp>"
  Bus Selector24/3 -> Mux29/2  "<BMS_module2Cell17Temp>"
  Bus Selector24/4 -> Mux29/3  "<BMS_module2Cell18Temp>"
  Bus Selector24/5 -> [IO_CAN2_526_cnt]  "<BMS_counterMsg526>"
  Bus Selector38/2 -> Mux36/1  "<BMS_module3Cell1Temp>"
  Bus Selector38/3 -> Mux36/2  "<BMS_module3Cell2Temp>"
  Bus Selector38/4 -> Mux36/3  "<BMS_module3Cell3Temp>"
  Bus Selector38/5 -> [IO_CAN2_533_cnt]  "<BMS_counterMsg533>"
  Bus Selector38/1 -> [IO_CAN2_533_Age]  "<Age>"
  [IO_CAN2_504_Age] -> Mux2/5
  OverMeas120/1 -> ?  "IN_module4Cell5V_V"
  OverMeas132/1 -> ?  "IN_module4Cell14V_V"
  OverMeas119/1 -> ?  "IN_module4Cell4V_V"
  OverMeas131/1 -> ?  "IN_module4Cell12V_V"
  OverMeas123/1 -> ?  "IN_module4Cell8V_V"
  OverMeas121/1 -> ?  "IN_module4Cell6V_V"
  OverMeas124/1 -> ?  "IN_module4Cell9V_V"
  OverMeas122/1 -> ?  "IN_module4Cell7V_V"
  OverMeas133/1 -> ?  "IN_module4Cell16V_V"
  OverMeas130/1 -> ?  "IN_module4Cell13V_V"
  Constant39/1 -> Switch39/1
  [IN_CAN2_543_Fault] -> Switch43/2
  Demux43/2 -> OverMeas129/1
  Demux44/2 -> OverMeas120/1
  [IN_CAN2_544_Fault] -> Switch44/2
  IO_CAN2_540_Bus/1 -> Bus Selector40/1  "IO_CAN2_540_Bus"
  Mux45/1 -> Switch40/3
  Mux43/1 -> Switch43/3
  Mux44/1 -> Switch44/3
  OverMeas126/1 -> ?  "IN_module4Cell17V_V"
  [IN_CAN2_542_Fault] -> Switch42/2
  Demux43/3 -> OverMeas131/1
  Demux46/2 -> OverMeas132/1
  IO_CAN2_544_Bus/1 -> Bus Selector44/1  "IO_CAN2_544_Bus"
  Demux46/1 -> OverMeas130/1
  [IN_CAN2_539_Fault] -> Switch39/2
  Demux42/1 -> OverMeas133/1
  [IN_CAN2_540_Fault] -> Switch40/2
  IO_CAN2_542_Bus/1 -> Bus Selector42/1  "IO_CAN2_542_Bus"
  Mux42/1 -> Switch39/3
  Demux43/1 -> OverMeas128/1
  Demux41/2 -> OverMeas116/1
  IO_CAN2_543_Bus/1 -> Bus Selector43/1  "IO_CAN2_543_Bus"
  Demux41/1 -> OverMeas118/1
  Switch40/1 -> Demux44/1
  Demux44/1 -> OverMeas119/1
  Switch42/1 -> Demux43/1
  Constant41/1 -> Switch41/1
  Demux44/3 -> OverMeas121/1
  Demux42/3 -> OverMeas127/1
  Demux46/3 -> OverMeas125/1
  Demux45/3 -> OverMeas124/1
  Switch44/1 -> Demux42/1
  Mux47/1 -> Switch42/3
  Constant44/1 -> Switch44/1
  Bus Selector10/1 -> [IO_CAN2_539_Age]  "<Age>"
  Mux46/1 -> Switch41/3
  OverMeas125/1 -> ?  "IN_module4Cell15V_V"
  Demux41/3 -> OverMeas117/1
  Switch39/1 -> Demux41/1
  Constant43/1 -> Switch43/1
  Demux45/2 -> OverMeas123/1
  Constant40/1 -> Switch40/1
  Demux45/1 -> OverMeas122/1
  IO_CAN2_539_Bus/1 -> Bus Selector10/1  "IO_CAN2_539_Bus"
  OverMeas129/1 -> ?  "IN_module4Cell11V_V"
  Demux42/2 -> OverMeas126/1
  OverMeas128/1 -> ?  "IN_module4Cell10V_V"
  Constant42/1 -> Switch42/1
  OverMeas127/1 -> ?  "IN_module4Cell18V_V"
  [IN_CAN2_541_Fault] -> Switch41/2
  Switch41/1 -> Demux45/1
  OverMeas117/1 -> ?  "IN_module4Cell3V_V"
  OverMeas118/1 -> ?  "IN_module4Cell1V_V"
  Switch43/1 -> Demux46/1
  OverMeas116/1 -> ?  "IN_module4Cell2V_V"
  Bus Selector10/2 -> Mux42/1  "<BMS_module4Cell1Volt>"
  Bus Selector10/3 -> Mux42/2  "<BMS_module4Cell2Volt>"
  Bus Selector10/4 -> Mux42/3  "<BMS_module4Cell3Volt>"
  Bus Selector10/5 -> [IO_CAN2_539_cnt]  "<BMS_counterMsg539>"
  Bus Selector40/2 -> Mux45/1  "<BMS_module4Cell4Volt>"
  Bus Selector40/3 -> Mux45/2  "<BMS_module4Cell5Volt>"
  Bus Selector40/4 -> Mux45/3  "<BMS_module4Cell6Volt>"
  Bus Selector40/1 -> [IO_CAN2_540_Age]  "<Age>"
  Bus Selector40/5 -> [IO_CAN2_540_cnt]  "<BMS_counterMsg540>"
  IO_CAN2_541_Bus/1 -> Bus Selector41/1  "IO_CAN2_541_Bus"
  Bus Selector41/2 -> Mux46/1  "<BMS_module4Cell7Volt>"
  Bus Selector41/3 -> Mux46/2  "<BMS_module4Cell8Volt>"
  Bus Selector41/4 -> Mux46/3  "<BMS_module4Cell9Volt>"
  Bus Selector41/1 -> [IO_CAN2_541_Age]  "<Age>"
  Bus Selector41/5 -> [IO_CAN2_541_cnt]  "<BMS_counterMsg541>"
  Bus Selector42/2 -> Mux47/1  "<BMS_module4Cell10Volt>"
  Bus Selector42/3 -> Mux47/2  "<BMS_module4Cell11Volt>"
  Bus Selector42/4 -> Mux47/3  "<BMS_module4Cell12Volt>"
  Bus Selector42/1 -> [IO_CAN2_542_Age]  "<Age>"
  Bus Selector42/5 -> [IO_CAN2_542_cnt]  "<BMS_counterMsg542>"
  Bus Selector43/2 -> Mux43/1  "<BMS_module4Cell13Volt>"
  Bus Selector43/3 -> Mux43/2  "<BMS_module4Cell14Volt>"
  Bus Selector43/4 -> Mux43/3  "<BMS_module4Cell15Volt>"
  Bus Selector43/5 -> [IO_CAN2_543_cnt]  "<BMS_counterMsg543>"
  Bus Selector43/1 -> [IO_CAN2_543_Age]  "<Age>"
  Bus Selector45/1 -> [IO_CAN2_546_Age]  "<Age>"
  Demux50/2 -> OverMeas145/1
  Demux50/1 -> OverMeas142/1
  OverMeas135/1 -> ?  "IN_module4Cell3Temp_degC"
  OverMeas147/1 -> ?  "IN_module4Cell15Temp_degC"
  OverMeas142/1 -> ?  "IN_modul4Cell13Temp_degC"
  Switch48/1 -> Demux50/1
  Switch47/1 -> Demux52/1
  IO_CAN2_549_Bus/1 -> Bus Selector49/1  "IO_CAN2_549_Bus"
  Constant48/1 -> Switch48/1
  Mux52/1 -> Switch47/3
  Demux51/3 -> OverMeas149/1
  [IN_CAN2_547_Fault] -> Switch46/2
  Demux48/3 -> OverMeas138/1
  Demux52/2 -> OverMeas144/1
  Demux48/2 -> OverMeas137/1
  [IN_CAN2_548_Fault] -> Switch47/2
  IO_CAN2_546_Bus/1 -> Bus Selector45/1  "IO_CAN2_546_Bus"
  Demux49/2 -> OverMeas140/1
  Switch49/1 -> Demux51/1
  Switch45/1 -> Demux48/1
  Mux51/1 -> Switch46/3
  Demux49/1 -> OverMeas139/1
  Constant47/1 -> Switch47/1
  Switch46/1 -> Demux49/1
  Demux47/3 -> OverMeas135/1
  [IN_CAN2_534_Fault] -> Switch45/2
  [IN_CAN2_549_Fault] -> Switch48/2
  Demux52/1 -> OverMeas143/1
  OverMeas139/1 -> ?  "IN_module4Cell7Temp_degC"
  Constant46/1 -> Switch46/1
  OverMeas151/1 -> ?  "IN_module4Cell1Temp_degC"
  Demux48/1 -> OverMeas136/1
  [IN_CAN2_550_Fault] -> Switch49/2
  OverMeas141/1 -> ?  "IN_module4Cell9Temp_degC"
  Demux52/3 -> OverMeas146/1
  OverMeas134/1 -> ?  "IN_module4Cell2Temp_degC"
  Constant45/1 -> Switch45/1
  OverMeas137/1 -> ?  "IN_module4Cell5Temp_degC"
  Demux50/3 -> OverMeas147/1
  Mux48/1 -> Switch50/3
  Demux49/3 -> OverMeas141/1
  OverMeas138/1 -> ?  "IN_module4Cell6Temp_degC"
  Mux50/1 -> Switch45/3
  OverMeas144/1 -> ?  "IN_module4Cell11Temp_degC"
  OverMeas146/1 -> ?  "IN_module4Cell12Temp_degC"
  OverMeas143/1 -> ?  "IN_module4Cell10Temp_degC"
  OverMeas150/1 -> ?  "IN_module4Cell16Temp_degC"
  OverMeas140/1 -> ?  "IN_module4Cell8Temp_degC"
  Demux51/2 -> OverMeas148/1
  Demux51/1 -> OverMeas150/1
  Mux49/1 -> Switch48/3
  Constant49/1 -> Switch49/1
  Mux53/1 -> Switch49/3
  OverMeas148/1 -> ?  "IN_module4Cell17Temp_degC"
  Switch50/1 -> Demux47/1
  Constant50/1 -> Switch50/1
  [IN_CAN2_545_Fault] -> Switch50/2
  OverMeas136/1 -> ?  "IN_module4Cell4Temp_degC"
  Demux47/2 -> OverMeas134/1
  Demux47/1 -> OverMeas151/1
  OverMeas145/1 -> ?  "IN_module4Cell14Temp_degC"
  OverMeas149/1 -> ?  "IN_module4Cell18Temp_degC"
  IO_CAN2_550_Bus/1 -> Bus Selector48/1  "IO_CAN2_550_Bus"
  IO_CAN2_547_Bus/1 -> Bus Selector46/1  "IO_CAN2_547_Bus"
  IO_CAN2_545_Bus/1 -> Bus Selector50/1  "IO_CAN2_545_Bus"
  IO_CAN2_548_Bus/1 -> Bus Selector47/1  "IO_CAN2_548_Bus"
  Bus Selector50/1 -> [IO_CAN2_545_Age]  "<Age>"
  Bus Selector50/2 -> Mux48/1  "<BMS_module4Cell1Temp>"
  Bus Selector50/3 -> Mux48/2  "<BMS_module4Cell2Temp>"
  Bus Selector50/4 -> Mux48/3  "<BMS_module4Cell3Temp>"
  Bus Selector50/5 -> [IO_CAN2_545_cnt]  "<BMS_counterMsg545>"
  Bus Selector45/2 -> Mux50/1  "<BMS_module4Cell4Temp>"
  Bus Selector45/3 -> Mux50/2  "<BMS_module4Cell5Temp>"
  Bus Selector45/4 -> Mux50/3  "<BMS_module4Cell6Temp>"
  Bus Selector45/5 -> [IO_CAN2_546_cnt]  "<BMS_counterMsg546>"
  Bus Selector46/1 -> [IO_CAN2_547_Age]  "<Age>"
  Bus Selector46/2 -> Mux51/1  "<BMS_module4Cell7Temp>"
  Bus Selector46/3 -> Mux51/2  "<BMS_module4Cell8Temp>"
  Bus Selector46/4 -> Mux51/3  "<BMS_module4Cell9Temp>"
  Bus Selector46/5 -> [IO_CAN2_547_cnt]  "<BMS_counterMsg547>"
  Bus Selector47/1 -> [IO_CAN2_548_Age]  "<Age>"
  Bus Selector47/2 -> Mux52/1  "<BMS_module4Cell10Temp>"
  Bus Selector47/3 -> Mux52/2  "<BMS_module4Cell11Temp>"
  Bus Selector47/4 -> Mux52/3  "<BMS_module4Cell12Temp>"
  Bus Selector47/5 -> [IO_CAN2_548_cnt]  "<BMS_counterMsg548>"
  Bus Selector49/2 -> Mux49/1  "<BMS_module4Cell13Temp>"
  Bus Selector49/3 -> Mux49/2  "<BMS_module4Cell14Temp>"
  Bus Selector49/4 -> Mux49/3  "<BMS_module4Cell15Temp>"
  Bus Selector49/5 -> [IO_CAN2_549_cnt]  "<BMS_counterMsg549>"
  Bus Selector49/1 -> [IO_CAN2_549_Age]  "<Age>"
  Bus Selector48/2 -> Mux53/1  "<BMS_module4Cell16Temp>"
  Bus Selector48/3 -> Mux53/2  "<BMS_module4Cell17Temp>"
  Bus Selector48/4 -> Mux53/3  "<BMS_module4Cell18Temp>"
  Bus Selector48/5 -> [IO_CAN2_550_cnt]  "<BMS_counterMsg550>"
  Bus Selector48/1 -> [IO_CAN2_550_Age]  "<Age>"
  Bus Selector44/5 -> [IO_CAN2_544_cnt]  "<BMS_counterMsg544>"
  Bus Selector44/4 -> Mux44/3  "<BMS_module4Cell18Volt>"
  Bus Selector44/3 -> Mux44/2  "<BMS_module4Cell17Volt>"
  Bus Selector44/2 -> Mux44/1  "<BMS_module4Cell16Volt>"
  Bus Selector44/1 -> [IO_CAN2_544_Age]  "<Age>"
  IO_CAN2_556_Bus/1 -> Bus Selector56/1  "IO_CAN2_556_Bus"
  IO_CAN2_552_Bus/1 -> Bus Selector52/1  "IO_CAN2_552_Bus"
  OverMeas167/1 -> ?  "IN_module5Cell12V_V"
  OverMeas152/1 -> ?  "IN_module5Cell2V_V"
  OverMeas154/1 -> ?  "IN_module5Cell1V_V"
  Constant54/1 -> Switch54/1
  OverMeas153/1 -> ?  "IN_module5Cell3V_V"
  Switch53/1 -> Demux57/1
  [IN_CAN2_553_Fault] -> Switch53/2
  IO_CAN2_555_Bus/1 -> Bus Selector55/1  "IO_CAN2_555_Bus"
  OverMeas164/1 -> ?  "IN_module5Cell10V_V"
  OverMeas165/1 -> ?  "IN_module5Cell11V_V"
  Demux57/1 -> OverMeas158/1
  Demux53/3 -> OverMeas153/1
  Constant55/1 -> Switch55/1
  OverMeas169/1 -> ?  "IN_module5Cell16V_V"
  OverMeas160/1 -> ?  "IN_module4Cell9V_V"
  Switch51/1 -> Demux53/1
  OverMeas157/1 -> ?  "IN_module5Cell6V_V"
  IO_CAN2_553_Bus/1 -> Bus Selector53/1  "IO_CAN2_553_Bus"
  OverMeas156/1 -> ?  "IN_module5Cell5V_V"
  OverMeas163/1 -> ?  "IN_module5Cell18V_V"
  Demux57/2 -> OverMeas159/1
  Constant51/1 -> Switch51/1
  Demux58/2 -> OverMeas168/1
  Demux55/3 -> OverMeas167/1
  Demux58/1 -> OverMeas166/1
  OverMeas159/1 -> ?  "IN_module5Cell8V_V"
  OverMeas155/1 -> ?  "IN_module5Cell4V_V"
  Switch55/1 -> Demux58/1
  OverMeas166/1 -> ?  "IN_module5Cell13V_V"
  [IN_CAN2_556_Fault] -> Switch56/2
  Demux54/2 -> OverMeas162/1
  Demux56/2 -> OverMeas156/1
  [IN_CAN2_554_Fault] -> Switch54/2
  Mux56/1 -> Switch56/3
  Mux55/1 -> Switch55/3
  Mux57/1 -> Switch52/3
  Demux57/3 -> OverMeas160/1
  Constant52/1 -> Switch52/1
  Switch56/1 -> Demux54/1
  Demux58/3 -> OverMeas161/1
  Demux55/2 -> OverMeas165/1
  Demux56/1 -> OverMeas155/1
  Switch54/1 -> Demux55/1
  OverMeas158/1 -> ?  "IN_module5Cell7V_V"
  Switch52/1 -> Demux56/1
  OverMeas168/1 -> ?  "IN_module5Cell14V_V"
  Demux56/3 -> OverMeas157/1
  Constant53/1 -> Switch53/1
  Demux54/3 -> OverMeas163/1
  Demux53/1 -> OverMeas154/1
  Demux53/2 -> OverMeas152/1
  Demux55/1 -> OverMeas164/1
  OverMeas162/1 -> ?  "IN_module5Cell17V_V"
  Mux54/1 -> Switch51/3
  OverMeas161/1 -> ?  "IN_module5Cell15V_V"
  IO_CAN2_554_Bus/1 -> Bus Selector54/1  "IO_CAN2_554_Bus"
  Constant56/1 -> Switch56/1
  Mux59/1 -> Switch54/3
  Demux54/1 -> OverMeas169/1
  IO_CAN2_551_Bus/1 -> Bus Selector51/1  "IO_CAN2_551_Bus"
  Mux58/1 -> Switch53/3
  [IN_CAN2_551_Fault] -> Switch51/2
  [IN_CAN2_552_Fault] -> Switch52/2
  [IN_CAN2_555_Fault] -> Switch55/2
  Bus Selector51/2 -> Mux54/1  "<BMS_module5Cell1Volt>"
  Bus Selector51/3 -> Mux54/2  "<BMS_module5Cell2Volt>"
  Bus Selector51/4 -> Mux54/3  "<BMS_module5Cell3Volt>"
  Bus Selector51/5 -> [IO_CAN2_551_cnt]  "<BMS_counterMsg551>"
  Bus Selector51/1 -> [IO_CAN2_551_Age]  "<Age>"
  Bus Selector52/2 -> Mux57/1  "<BMS_module5Cell4Volt>"
  Bus Selector52/3 -> Mux57/2  "<BMS_module5Cell5Volt>"
  Bus Selector52/4 -> Mux57/3  "<BMS_module5Cell6Volt>"
  Bus Selector52/5 -> [IO_CAN2_552_cnt]  "<BMS_counterMsg552>"
  Bus Selector52/1 -> [IO_CAN2_552_Age]  "<Age>"
  Bus Selector53/2 -> Mux58/1  "<BMS_module5Cell7Volt>"
  Bus Selector53/3 -> Mux58/2  "<BMS_module5Cell8Volt>"
  Bus Selector53/4 -> Mux58/3  "<BMS_module5Cell9Volt>"
  Bus Selector53/5 -> [IO_CAN2_553_cnt]  "<BMS_counterMsg553>"
  Bus Selector53/1 -> [IO_CAN2_553_Age]  "<Age>"
  Bus Selector54/2 -> Mux59/1  "<BMS_module5Cell10Volt>"
  Bus Selector54/3 -> Mux59/2  "<BMS_module5Cell11Volt>"
  Bus Selector54/4 -> Mux59/3  "<BMS_module5Cell12Volt>"
  Bus Selector54/5 -> [IO_CAN2_554_cnt]  "<BMS_counterMsg554>"
  Bus Selector54/1 -> [IO_CAN2_554_Age]  "<Age>"
  Bus Selector55/1 -> [IO_CAN2_555_Age]  "<Age>"
  Bus Selector55/2 -> Mux55/1  "<BMS_module5Cell13Volt>"
  Bus Selector55/3 -> Mux55/2  "<BMS_module5Cell14Volt>"
  Bus Selector55/4 -> Mux55/3  "<BMS_module5Cell15Volt>"
  Bus Selector55/5 -> [IO_CAN2_555_cnt]  "<BMS_counterMsg555>"
  Bus Selector56/5 -> [IO_CAN2_556_cnt]  "<BMS_counterMsg556>"
  Bus Selector56/1 -> [IO_CAN2_556_Age]  "<Age>"
  Bus Selector56/2 -> Mux56/1  "<BMS_module5Cell16Volt>"
  Bus Selector56/3 -> Mux56/2  "<BMS_module5Cell17Volt>"
  Bus Selector56/4 -> Mux56/3  "<BMS_module5Cell18Volt>"
  IO_CAN2_560_Bus/1 -> Bus Selector59/1  "IO_CAN2_560_Bus"
  IO_CAN2_561_Bus/1 -> Bus Selector61/1  "IO_CAN2_561_Bus"
  In63/1 -> Bus Selector60/1  "IO_CAN2_550_Bus"
  Constant60/1 -> Switch60/1
  Switch60/1 -> Demux62/1
  Switch59/1 -> Demux64/1
  OverMeas178/1 -> ?  "IN_module5Cell13Temp_degC"
  OverMeas171/1 -> ?  "IN_module4Cell3Temp_degC"
  Bus Selector57/1 -> [IO_CAN2_558_Age]  "<Age>"
  Demux62/2 -> OverMeas181/1
  OverMeas183/1 -> ?  "IN_module5Cell15Temp_degC"
  Demux62/1 -> OverMeas178/1
  Mux65/1 -> Switch61/3
  Constant61/1 -> Switch61/1
  Mux61/1 -> Switch60/3
  Demux63/2 -> OverMeas184/1
  OverMeas186/1 -> ?  "IN_module5Cell16Temp_degC"
  OverMeas182/1 -> ?  "IN_module5Cell12Temp_degC"
  Mux62/1 -> Switch57/3
  OverMeas179/1 -> ?  "IN_module5Cell10Temp_degC"
  IO_CAN2_558_Bus/1 -> Bus Selector57/1  "IO_CAN2_558_Bus"
  OverMeas176/1 -> ?  "IN_module5Cell8Temp_degC"
  OverMeas174/1 -> ?  "IN_module4Cell6Temp_degC"
  Demux62/3 -> OverMeas183/1
  OverMeas173/1 -> ?  "IN_module4Cell5Temp_degC"
  Demux61/3 -> OverMeas177/1
  Mux60/1 -> Switch62/3
  [IN_CAN2_562_Fault] -> Switch61/2
  OverMeas177/1 -> ?  "IN_module5Cell9Temp_degC"
  Demux61/1 -> OverMeas175/1
  [IN_CAN2_561_Fault] -> Switch60/2
  Demux59/3 -> OverMeas171/1
  OverMeas175/1 -> ?  "IN_module5Cell7Temp_degC"
  [IN_CAN2_558_Fault] -> Switch57/2
  Constant59/1 -> Switch59/1
  Demux60/1 -> OverMeas172/1
  Switch57/1 -> Demux60/1
  Demux64/2 -> OverMeas180/1
  Demux63/3 -> OverMeas185/1
  [IN_CAN2_559_Fault] -> Switch58/2
  Demux61/2 -> OverMeas176/1
  Switch61/1 -> Demux63/1
  OverMeas180/1 -> ?  "IN_module5Cell11Temp_degC"
  OverMeas185/1 -> ?  "IN_module5Cell18Temp_degC"
  Demux60/3 -> OverMeas174/1
  Demux59/2 -> OverMeas170/1
  OverMeas181/1 -> ?  "IN_module5Cell14Temp_degC"
  OverMeas172/1 -> ?  "IN_module4Cell4Temp_degC"
  Constant62/1 -> Switch62/1
  [IN_CAN2_557_Fault] -> Switch62/2
  Demux63/1 -> OverMeas186/1
  Switch62/1 -> Demux59/1
  Mux64/1 -> Switch59/3
  OverMeas170/1 -> ?  "IN_module4Cell2Temp_degC"
  Demux64/3 -> OverMeas182/1
  Constant58/1 -> Switch58/1
  [IN_CAN2_560_Fault] -> Switch59/2
  Demux60/2 -> OverMeas173/1
  Switch58/1 -> Demux61/1
  OverMeas184/1 -> ?  "IN_module5Cell17Temp_degC"
  Mux63/1 -> Switch58/3
  OverMeas187/1 -> ?  "IN_module4Cell1Temp_degC"
  Demux59/1 -> OverMeas187/1
  Demux64/1 -> OverMeas179/1
  Constant57/1 -> Switch57/1
  IO_CAN2_559_Bus/1 -> Bus Selector58/1  "IO_CAN2_559_Bus"
  IO_CAN2_557_Bus/1 -> Bus Selector62/1  "IO_CAN2_557_Bus"
  Bus Selector62/1 -> [IO_CAN2_557_Age]  "<Age>"
  Bus Selector62/2 -> Mux60/1  "<BMS_module5Cell1Temp>"
  Bus Selector62/3 -> Mux60/2  "<BMS_module5Cell2Temp>"
  Bus Selector62/4 -> Mux60/3  "<BMS_module5Cell3Temp>"
  Bus Selector62/5 -> [IO_CAN2_557_cnt]  "<BMS_counterMsg557>"
  Bus Selector57/2 -> Mux62/1  "<BMS_module5Cell4Temp>"
  Bus Selector57/3 -> Mux62/2  "<BMS_module5Cell5Temp>"
  Bus Selector57/4 -> Mux62/3  "<BMS_module5Cell6Temp>"
  Bus Selector57/5 -> [IO_CAN2_558_cnt]  "<BMS_counterMsg558>"
  Bus Selector58/1 -> [IO_CAN2_559_Age]  "<Age>"
  Bus Selector58/2 -> Mux63/1  "<BMS_module5Cell7Temp>"
  Bus Selector58/3 -> Mux63/2  "<BMS_module5Cell8Temp>"
  Bus Selector58/4 -> Mux63/3  "<BMS_module5Cell9Temp>"
  Bus Selector58/5 -> [IO_CAN2_559_cnt]  "<BMS_counterMsg559>"
  Bus Selector59/1 -> [IO_CAN2_560_Age]  "<Age>"
  Bus Selector59/2 -> Mux64/1  "<BMS_module5Cell10Temp>"
  Bus Selector59/3 -> Mux64/2  "<BMS_module5Cell11Temp>"
  Bus Selector59/4 -> Mux64/3  "<BMS_module5Cell12Temp>"
  Bus Selector59/5 -> [IO_CAN2_560_cnt]  "<BMS_counterMsg560>"
  Bus Selector61/5 -> [IO_CAN2_561_cnt]  "<BMS_counterMsg561>"
  Bus Selector61/4 -> Mux61/3  "<BMS_module5Cell15Temp>"
  Bus Selector61/3 -> Mux61/2  "<BMS_module5Cell14Temp>"
  Bus Selector61/2 -> Mux61/1  "<BMS_module5Cell13Temp>"
  Bus Selector61/1 -> [IO_CAN2_561_Age]  "<Age>"
  Bus Selector60/1 -> [IO_CAN2_562_Age]  "<Age>"
  Bus Selector60/2 -> Mux65/1  "<BMS_module5Cell16Temp>"
  Bus Selector60/3 -> Mux65/2  "<BMS_module5Cell17Temp>"
  Bus Selector60/4 -> Mux65/3  "<BMS_module5Cell18Temp>"
  Bus Selector60/5 -> [IO_CAN2_562_cnt]  "<BMS_counterMsg562>"
